simulink model "IEEE123bus_v2019b_Discrete"  (R2019b)
settings: Solver=ode4  StartTime=0.0  StopTime=5  FixedStep=Ts  MaxStep=1e-4  RelTol=1e-3
InitFcn:
  | a=1; % Loading Factor
  | Ts=50e-6;
  | % phase to sequence conversion of RXB matrices
  | c=1*exp(sqrt(-1)*(120*pi/180));
  | T=[1 1 1;1 c*c c;1 c c*c];
  | Tinv=1/3*[1 1 1;1 c c*c;1 c*c c];
  | 
  | % Simulation data for the IEEE 123 Node Test Feeder model
  | mi2km = 1.60934;%  miles to km conversion
  | ft2km = 0.0003048; % feet to km conversion
  | ms2F = 1*1e-6/(2*pi*60);% microsiemens to Farads conversion
  | 
  | %% Configuration 1
  | % Series Resitance and Reactance - ohm/mile
  | R_1 = [0.4576 0.1560 0.1535;0.1560 0.4666 0.1580;0.1535 0.1580 0.4615];
  | X_1 = [1.0780 0.5017 0.3849;0.5017 1.0482 0.4236;0.3849 0.4236 1.0651];
  | % charging susceptance - microsiemens/mile
  | B_1 = [5.6765 -1.8319 -0.6982;-1.8319 5.9809 -1.1645;-0.6982 -1.1645 5.3971];
  | 
  | R_1 = R_1/mi2km;
  | Rseq=Tinv*R_1*T;
  | R1_1=Rseq(2,2);R0_1=Rseq(1,1);
  | 
  | L_1 = (X_1/(2*pi*60))/mi2km;
  | Lseq=Tinv*L_1*T;
  | L1_1=Lseq(2,2);L0_1=Lseq(1,1);
  | 
  | C_1 =(B_1*ms2F)/mi2km;
  | Cseq=Tinv*C_1*T;
  | C1_1=Cseq(2,2);C0_1=Cseq(1,1);
  | %% Configuration 2 - series reactance - ohm/mile
  | R_2 = [0.4666 0.1580 0.1560;0.1580 0.4615 0.1535;0.1560 0.1535 0.4576];
  | X_2 = [1.0482 0.4236 0.5017;0.4236 1.0651 0.3849;0.5017 0.3849 1.0780];
  | % charging susceptance - microsiemens/mile
  | B_2 = [5.9809 -1.1645 -1.8319;-1.1645 5.3971 -0.6982;-1.8319 -0.6982 5.6765];
  | 
  | R_2 = R_2/mi2km;
  | Rseq=Tinv*R_2*T;
  | R1_2=Rseq(2,2);R0_2=Rseq(1,1);
  | 
  | L_2 = (X_2/(2*pi*60))/mi2km;
  | Lseq=Tinv*L_2*T;
  | L1_2=Lseq(2,2);L0_2=Lseq(1,1);
  | 
  | C_2 =(B_2*ms2F)/mi2km;
  | Cseq=Tinv*C_2*T;
  | C1_2=Cseq(2,2);C0_2=Cseq(1,1);
  | %% Configuration 3 - series reactance - ohm/mile
  | R_3 = [0.4615 0.1535 0.1580;0.1535 0.4576 0.1560;0.1580 0.1560 0.4666];
  | X_3 = [1.0651 0.3849 0.4236;0.3849 1.0780 0.5017;0.4236 0.5017 1.0482];
  | % charging susceptance - microsiemens/mile
  | B_3 = [5.3971 -0.6982 -1.1645;-0.6982 5.6765 -1.8319; -1.1645 -1.8319 5.9809];
  | 
  | R_3 = R_3/mi2km;
  | Rseq=Tinv*R_3*T;
  | R1_3=Rseq(2,2);R0_3=Rseq(1,1);
  | 
  | L_3 = (X_3/(2*pi*60))/mi2km;
  | Lseq=Tinv*L_3*T;
  | L1_3=Lseq(2,2);L0_3=Lseq(1,1);
  | 
  | C_3 =(B_3*ms2F)/mi2km;
  | Cseq=Tinv*C_3*T;
  | C1_3=Cseq(2,2);C0_3=Cseq(1,1);
  | %% Configuration 4 - series reactance - ohm/mile
  | R_4 = [0.4615 0.1580 0.1535;0.1580 0.4666 0.1560;0.1535 0.1560 0.4576];
  | X_4 = [1.0651 0.4236 0.3849;0.4236 1.0482 0.5017;0.3849 0.5017 1.0780];
  | % charging susceptance - microsiemens/mile
  | B_4 = [5.3971 -1.1645 -0.6982;-1.1645 5.9809 -1.8319;-0.6982 -1.8319 5.6765];
  | 
  | R_4 = R_4/mi2km;
  | Rseq=Tinv*R_4*T;
  | R1_4=Rseq(2,2);R0_4=Rseq(1,1);
  | 
  | L_4 = (X_4/(2*pi*60))/mi2km;
  | Lseq=Tinv*L_4*T;
  | L1_4=Lseq(2,2);L0_4=Lseq(1,1);
  | 
  | C_4 =(B_4*ms2F)/mi2km;
  | Cseq=Tinv*C_4*T;
  | C1_4=Cseq(2,2);C0_4=Cseq(1,1);
  | %% Configuration 5 - series reactance - ohm/mile
  | R_5 = [0.4666 0.1560 0.1580;0.1560 0.4576 0.1535;0.1580 0.1535 0.4615];
  | X_5 = [1.0482 0.5017 0.4236;0.5017 1.0780 0.3849;0.4236 0.3849 1.0651];
  | % charging susceptance - microsiemens/mile
  | B_5 = [5.9809 -1.8319 -1.1645;-1.8319 5.6765 -0.6982;-1.1645 -0.6982 5.3971];
  | 
  | R_5 = R_5/mi2km;
  | Rseq=Tinv*R_5*T;
  | R1_5=Rseq(2,2);R0_5=Rseq(1,1);
  | 
  | L_5 = (X_5/(2*pi*60))/mi2km;
  | Lseq=Tinv*L_5*T;
  | L1_5=Lseq(2,2);L0_5=Lseq(1,1);
  | 
  | C_5 =(B_5*ms2F)/mi2km;
  | Cseq=Tinv*C_5*T;
  | C1_5=Cseq(2,2);C0_5=Cseq(1,1);
  | %% Configuration 6 - series reactance - ohm/mile
  | R_6 = [0.4576 0.1535 0.1560;0.1535 0.4615 0.1580;0.1560 0.1580 0.4666];
  | X_6 = [1.0780 0.3849 0.5017;0.3849 1.0651 0.4236;0.5017 0.4236 1.0482];
  | % charging susceptance - microsiemens/mile
  | B_6 = [5.6765 -0.6982 -1.8319;-0.6982 5.3971 -1.1645;-1.8319 -1.1645 5.9809];
  | 
  | R_6 = R_6/mi2km;
  | Rseq=Tinv*R_6*T;
  | R1_6=Rseq(2,2);R0_6=Rseq(1,1);
  | 
  | L_6 = (X_6/(2*pi*60))/mi2km;
  | Lseq=Tinv*L_6*T;
  | L1_6=Lseq(2,2);L0_6=Lseq(1,1);
  | 
  | C_6 =(B_6*ms2F)/mi2km;
  | Cseq=Tinv*C_6*T;
  | C1_6=Cseq(2,2);C0_6=Cseq(1,1);
  | %% Configuration 7 - series reactance - ohm/mile
  | R_7 = [0.4576 0.0000 0.1535;0.0000 0.0000 0.0000;0.1535 0.0000 0.4615];
  | X_7 = [1.0780 0.0000 0.3849;0.0000 0.0000 0.0000;0.3849 0.0000 1.0651];
  | % charging susceptance - microsiemens/mile
  | B_7 = [5.1154 0.0000 -1.0549;0.0000 0.0000 0.0000;-1.0549 0.0000 5.1704];
  | 
  | R_7 = R_7/mi2km;
  | Rseq=Tinv*R_7*T;
  | R1_7=Rseq(2,2);R0_7=Rseq(1,1);
  | 
  | L_7 = (X_7/(2*pi*60))/mi2km;
  | Lseq=Tinv*L_7*T;
  | L1_7=Lseq(2,2);L0_7=Lseq(1,1);
  | 
  | C_7 =(B_7*ms2F)/mi2km;
  | Cseq=Tinv*C_7*T;
  | C1_7=Cseq(2,2);C0_7=Cseq(1,1);
  | %% Configuration 8 - series reactance - ohm/mile
  | R_8 = [0.4576 0.1535 0.0000;0.1535 0.4615 0.0000;0.0000 0.0000 0.0000];
  | X_8 = [1.0780 0.3849 0.0000;0.3849 1.0651 0.0000;0.0000 0.0000 0.0000];
  | % charging susceptance - microsiemens/mile
  | B_8 = [5.1154 -1.0549 0.0000;-1.0549 5.1704 0.0000;0.0000 0.0000 0.0000];
  | 
  | R_8 = R_8/mi2km;
  | Rseq=Tinv*R_8*T;
  | R1_8=Rseq(2,2);R0_8=Rseq(1,1);
  | 
  | L_8 = (X_8/(2*pi*60))/mi2km;
  | Lseq=Tinv*L_8*T;
  | L1_8=Lseq(2,2);L0_8=Lseq(1,1);
  | 
  | C_8 =(B_8*ms2F)/mi2km;
  | Cseq=Tinv*C_8*T;
  | C1_8=Cseq(2,2);C0_8=Cseq(1,1);
  | %% Configuration 9 - series reactance - ohm/mile
  | R_9 = [1.3292 0 0;0 0 0;0 0 0];
  | X_9 = [1.3475 0 0;0 0 0;0 0 0];
  | % charging susceptance - microsiemens/mile
  | B_9 = [4.5193 0 0;0 0 0;0 0 0];
  | 
  | R_9 = R_9/mi2km;
  | Rseq=Tinv*R_9*T;
  | R1_9=Rseq(2,2);R0_9=Rseq(1,1);
  | 
  | L_9 = (X_9/(2*pi*60))/mi2km;
  | Lseq=Tinv*L_9*T;
  | L1_9=Lseq(2,2);L0_9=Lseq(1,1);
  | 
  | C_9 =(B_9*ms2F)/mi2km;
  | Cseq=Tinv*C_9*T;
  | C1_9=Cseq(2,2);C0_9=Cseq(1,1);
  | %% Configuration 10- series reactance - ohm/mile
  | R_10 = [0 0 0;0 1.3292 0;0 0 0];
  | X_10 = [0 0 0;0 1.3475 0;0 0 0];
  | % charging susceptance - microsiemens/mile
  | B_10 = [0 0 0;0 4.5193 0;0 0 0];
  | 
  | R_10 = R_10/mi2km;
  | Rseq=Tinv*R_10*T;
  | R1_10=Rseq(2,2);R0_10=Rseq(1,1);
  | 
  | L_10 = (X_10/(2*pi*60))/mi2km;
  | Lseq=Tinv*L_10*T;
  | L1_10=Lseq(2,2);L0_10=Lseq(1,1);
  | 
  | C_10 =(B_10*ms2F)/mi2km;
  | Cseq=Tinv*C_10*T;
  | C1_10=Cseq(2,2);C0_10=Cseq(1,1);
  | %% Configuration 11 - series reactance - ohm/mile
  | R_11 = [0 0 0;0 0 0;0 0 1.3292];
  | X_11 = [0 0 0;0 0 0;0 0 1.3475];
  | % charging susceptance - microsiemens/mile
  | B_11 = [0 0 0;0 0 0;0 0 4.5193];
  | 
  | R_11 = R_11/mi2km;
  | Rseq=Tinv*R_11*T;
  | R1_11=Rseq(2,2);R0_11=Rseq(1,1);
  | 
  | L_11 = (X_11/(2*pi*60))/mi2km;
  | Lseq=Tinv*L_11*T;
  | L1_11=Lseq(2,2);L0_11=Lseq(1,1);
  | 
  | C_11 =(B_11*ms2F)/mi2km;
  | Cseq=Tinv*C_11*T;
  | C1_11=Cseq(2,2);C0_11=Cseq(1,1);
  | %% Configuration 12 - series reactance - ohm/mile
  | R_12 = [1.5209 0.5198 0.4924;0.5198 1.5329 0.5198;0.4924 0.5198 1.5209];
  | X_12 = [0.7521 0.2775 0.2157;0.2775 0.7162 0.2775;0.2157 0.2775 0.7521];
  | % charging susceptance - microsiemens/mile
  | B_12 = [67.2242 0.0000 0.0000;0.0000 67.2242 0.0000;0.0000 0.0000 67.2242];
  | 
  | R_12 = R_12/mi2km;
  | Rseq=Tinv*R_12*T;
  | R1_12=Rseq(2,2);R0_12=Rseq(1,1);
  | 
  | L_12 = (X_12/(2*pi*60))/mi2km;
  | Lseq=Tinv*L_12*T;
  | L1_12=Lseq(2,2);L0_12=Lseq(1,1);
  | 
  | C_12 =(B_12*ms2F)/mi2km;
  | Cseq=Tinv*C_12*T;
  | C1_12=Cseq(2,2);C0_12=Cseq(1,1);
undefined symbols (not defined in the file): D1, Delta, find_system
libraries: powerlib x768, powerlib_meascontrol x39
(part 1 of 6)
settings Model: ARTEMISmethode_block_infos=$$__separator__$$pi123variableloadwith3PV/ARTEMIS Guide$$__separator__$$  Creator=Arun  LastModifiedBy=USARSUR
settings DataIOCC: ReturnWorkspaceOutputs=off
settings DebuggingCC: UnconnectedInputMsg=none  UnconnectedOutputMsg=none  UnconnectedLineMsg=none  ArithmeticOperatorsInVariantConditions=warning
settings SFSimCC: SimUseLocalCustomCode=off  CustomCodeUndefinedFunction=UseInterfaceOnly
settings RTWCC: RTWUseLocalCustomCode=off
settings CodeAppCC: StateflowObjectComments=on
settings SimscapeCC: SimscapeNormalizeSystem=off

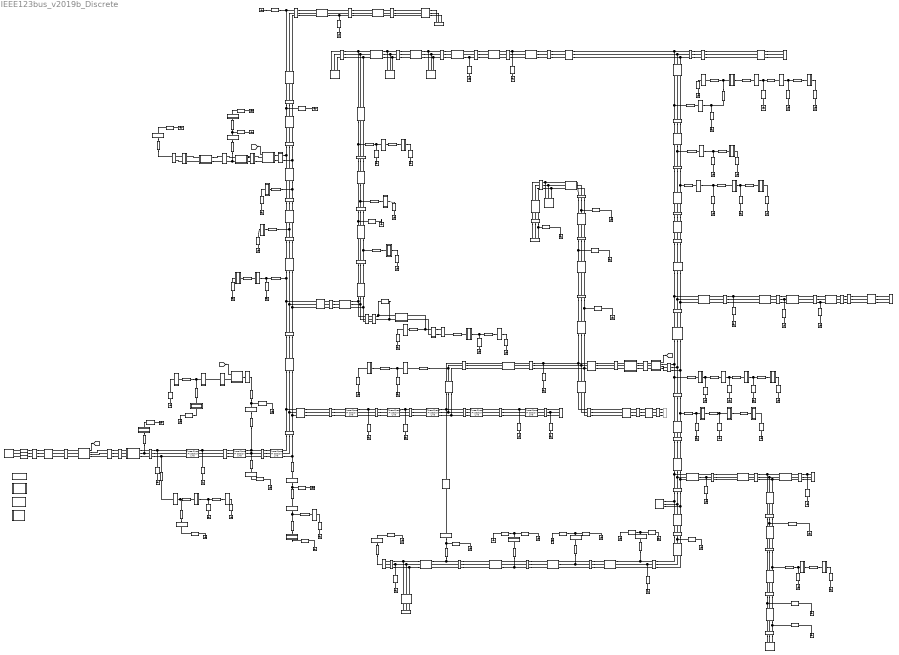
== system IEEE123bus_v2019b_Discrete ==
  note: Please consider citing following papers if the model was useful for your research
      |
      | A. Suresh, R. Bisht and S. Kamalasadan, "A Coordinated Control Architecture With Inverter-Based Resources and Legacy
      | Controllers of Power Distribution System for Voltage Profile Balance," in IEEE Transactions on Industry Applications, vol. 58,
      | no. 5, pp. 6701-6712, Sept.-Oct. 2022, doi: 10.1109/TIA.2022.3183030.
      |
      | A. Suresh, R. Bisht and S. Kamalasadan, "ADMM Based LQR for Voltage Regulation Using Distributed Energy Resources,"
      | 2020 IEEE International Conference on Power Electronics, Drives and Energy Systems (PEDES), 2020, pp. 1-6,
      | doi: 10.1109/PEDES49360.2020.9379625.
  note: Model Created by
      | Arun Suresh, Dr. Sukumar Kamalasadan,
      | University of North Carolina, Charlotte
  1 : powerlib/Measurements/Three-Phase V-I Measurement  VoltageMeasurement=phase-to-ground  SetLabelV=on  LabelV=V1  Vpu=off  VpuLL=off  CurrentMeasurement=no  SetLabelI=on  LabelI=I800  Ipu=off  Pbase=100e6  Vbase=24900  OutputType=Complex  PhasorSimulation=on  PSBequivalent=0
      settings: SourceProductName=Simscape Electrical
  1 Y PQ : powerlib/Elements/Series RLC Load  LConnTagsString=a  RConnTagsString=__new0  NominalVoltage=1.0*2401.78  NominalFrequency=60  ActivePower=40e3*a  InductivePower=20e3*a  CapacitivePower=0  Setx0=off  InitialVoltage=0  SetiL0=off  InitialCurrent=0  Measurements=None  LoadType=constant PQ
      settings: SourceProductName=Simscape Electrical
  1-2 10 : powerlib/Elements/Pi Section Line  LConnTagsString=__new0  RConnTagsString=__new0  Frequency=60  Resistance=R1_10  Inductance=L1_10  Capacitance=C1_10  Length=175*ft2km  PiSections=1  Measurements=None
      settings: AttributesFormatString=\n  SourceProductName=Simscape Electrical  SourceProductBaseCode=PS
  1-3 11 : powerlib/Elements/Pi Section Line  LConnTagsString=__new0  RConnTagsString=__new0  Frequency=60  Resistance=R1_11  Inductance=L1_11  Capacitance=C1_11  Length=250*ft2km  PiSections=1  Measurements=None
      settings: AttributesFormatString=\n  SourceProductName=Simscape Electrical  SourceProductBaseCode=PS
  1-7 1 : powerlib/Elements/Three-Phase PI Section Line  LConnTagsString=a|b|c  RConnTagsString=A|B|C  Frequency=60  Resistances=[R1_1 R0_1]  Inductances=[L1_1 L0_1]  Capacitances=[C1_1 C0_1]  Length=300*ft2km
      settings: SourceProductName=Simscape Electrical
  10 : Subsystem
  10 Y I : powerlib/Elements/Series RLC Load  LConnTagsString=a  RConnTagsString=__new0  NominalVoltage=1.0*2401.78  NominalFrequency=60  ActivePower=20e3*a  InductivePower=10e3*a  CapacitivePower=0  Setx0=off  InitialVoltage=0  SetiL0=off  InitialCurrent=0  Measurements=None  LoadType=constant I
      settings: SourceProductName=Simscape Electrical
  100 : powerlib/Measurements/Three-Phase V-I Measurement  VoltageMeasurement=phase-to-ground  SetLabelV=on  LabelV=V100  Vpu=off  VpuLL=off  CurrentMeasurement=no  SetLabelI=on  LabelI=I65  Ipu=off  Pbase=100e6  Vbase=24900  OutputType=Complex  PhasorSimulation=on  PSBequivalent=0
      settings: SourceProductName=Simscape Electrical
  100 Y Z : powerlib/Elements/Series RLC Load  LConnTagsString=a  RConnTagsString=__new0  NominalVoltage=1.0*2401.78  NominalFrequency=60  ActivePower=40e3*a  InductivePower=20e3*a  CapacitivePower=0  Setx0=off  InitialVoltage=0  SetiL0=off  InitialCurrent=0  Measurements=None  LoadType=constant Z
      settings: SourceProductName=Simscape Electrical
  100-450 3 : powerlib/Elements/Three-Phase PI Section Line  LConnTagsString=a|b|c  RConnTagsString=A|B|C  Frequency=60  Resistances=[R1_3 R0_3]  Inductances=[L1_3 L0_3]  Capacitances=[C1_3 C0_3]  Length=800*ft2km
      settings: SourceProductName=Simscape Electrical
  101 : powerlib/Measurements/Three-Phase V-I Measurement  VoltageMeasurement=phase-to-ground  SetLabelV=on  LabelV=V101  Vpu=off  VpuLL=off  CurrentMeasurement=no  SetLabelI=on  LabelI=I65  Ipu=off  Pbase=100e6  Vbase=24900  OutputType=Complex  PhasorSimulation=on  PSBequivalent=0
      settings: SourceProductName=Simscape Electrical
  101-102 11 : powerlib/Elements/Pi Section Line  LConnTagsString=__new0  RConnTagsString=__new0  Frequency=60  Resistance=R1_11  Inductance=L1_11  Capacitance=C1_11  Length=225*ft2km  PiSections=1  Measurements=None
      settings: AttributesFormatString=\n  SourceProductName=Simscape Electrical  SourceProductBaseCode=PS
  101-105 3 : powerlib/Elements/Three-Phase PI Section Line  LConnTagsString=a|b|c  RConnTagsString=A|B|C  Frequency=60  Resistances=[R1_3 R0_3]  Inductances=[L1_3 L0_3]  Capacitances=[C1_3 C0_3]  Length=275*ft2km
      settings: SourceProductName=Simscape Electrical
  102 : Subsystem
  102 Y Z : powerlib/Elements/Series RLC Load  LConnTagsString=a  RConnTagsString=__new0  NominalVoltage=1.0*2401.78  NominalFrequency=60  ActivePower=20e3*a  InductivePower=10e3*a  CapacitivePower=0  Setx0=off  InitialVoltage=0  SetiL0=off  InitialCurrent=0  Measurements=None  LoadType=constant Z
      settings: SourceProductName=Simscape Electrical
  102-103 11 : powerlib/Elements/Pi Section Line  LConnTagsString=__new0  RConnTagsString=__new0  Frequency=60  Resistance=R1_11  Inductance=L1_11  Capacitance=C1_11  Length=325*ft2km  PiSections=1  Measurements=None
      settings: AttributesFormatString=\n  SourceProductName=Simscape Electrical  SourceProductBaseCode=PS
  103 : Subsystem
  103 Y PQ : powerlib/Elements/Series RLC Load  LConnTagsString=a  RConnTagsString=__new0  NominalVoltage=1.0*2401.78  NominalFrequency=60  ActivePower=40e3*a  InductivePower=20e3*a  CapacitivePower=0  Setx0=off  InitialVoltage=0  SetiL0=off  InitialCurrent=0  Measurements=None  LoadType=constant PQ
      settings: SourceProductName=Simscape Electrical
  103-104 11 : powerlib/Elements/Pi Section Line  LConnTagsString=__new0  RConnTagsString=__new0  Frequency=60  Resistance=R1_11  Inductance=L1_11  Capacitance=C1_11  Length=700*ft2km  PiSections=1  Measurements=None
      settings: AttributesFormatString=\n  SourceProductName=Simscape Electrical  SourceProductBaseCode=PS
  104 : Subsystem
  104 Y PQ : powerlib/Elements/Series RLC Load  LConnTagsString=a  RConnTagsString=__new0  NominalVoltage=1.0*2401.78  NominalFrequency=60  ActivePower=40e3*a  InductivePower=20e3*a  CapacitivePower=0  Setx0=off  InitialVoltage=0  SetiL0=off  InitialCurrent=0  Measurements=None  LoadType=constant PQ
      settings: SourceProductName=Simscape Electrical
  105 : powerlib/Measurements/Three-Phase V-I Measurement  VoltageMeasurement=phase-to-ground  SetLabelV=on  LabelV=V105  Vpu=off  VpuLL=off  CurrentMeasurement=no  SetLabelI=on  LabelI=I65  Ipu=off  Pbase=100e6  Vbase=24900  OutputType=Complex  PhasorSimulation=on  PSBequivalent=0
      settings: SourceProductName=Simscape Electrical
  105-106 10 : powerlib/Elements/Pi Section Line  LConnTagsString=__new0  RConnTagsString=__new0  Frequency=60  Resistance=R1_10  Inductance=L1_10  Capacitance=C1_10  Length=225*ft2km  PiSections=1  Measurements=None
      settings: AttributesFormatString=\n  SourceProductName=Simscape Electrical  SourceProductBaseCode=PS
  105-108 3 : powerlib/Elements/Three-Phase PI Section Line  LConnTagsString=a|b|c  RConnTagsString=A|B|C  Frequency=60  Resistances=[R1_3 R0_3]  Inductances=[L1_3 L0_3]  Capacitances=[C1_3 C0_3]  Length=325*ft2km
      settings: SourceProductName=Simscape Electrical
  106 : Subsystem
  106 Y PQ : powerlib/Elements/Series RLC Load  LConnTagsString=a  RConnTagsString=__new0  NominalVoltage=1.0*2401.78  NominalFrequency=60  ActivePower=40e3*a  InductivePower=20e3*a  CapacitivePower=0  Setx0=off  InitialVoltage=0  SetiL0=off  InitialCurrent=0  Measurements=None  LoadType=constant PQ
      settings: SourceProductName=Simscape Electrical
  106-107 10 : powerlib/Elements/Pi Section Line  LConnTagsString=__new0  RConnTagsString=__new0  Frequency=60  Resistance=R1_10  Inductance=L1_10  Capacitance=C1_10  Length=575*ft2km  PiSections=1  Measurements=None
      settings: AttributesFormatString=\n  SourceProductName=Simscape Electrical  SourceProductBaseCode=PS
  107 : Subsystem
  107 Y PQ : powerlib/Elements/Series RLC Load  LConnTagsString=a  RConnTagsString=__new0  NominalVoltage=1.0*2401.78  NominalFrequency=60  ActivePower=40e3*a  InductivePower=20e3*a  CapacitivePower=0  Setx0=off  InitialVoltage=0  SetiL0=off  InitialCurrent=0  Measurements=None  LoadType=constant PQ
      settings: SourceProductName=Simscape Electrical
  108 : powerlib/Measurements/Three-Phase V-I Measurement  VoltageMeasurement=phase-to-ground  SetLabelV=on  LabelV=V108  Vpu=off  VpuLL=off  CurrentMeasurement=no  SetLabelI=on  LabelI=I65  Ipu=off  Pbase=100e6  Vbase=24900  OutputType=Complex  PhasorSimulation=on  PSBequivalent=0
      settings: SourceProductName=Simscape Electrical
  108-109 9 : powerlib/Elements/Pi Section Line  LConnTagsString=__new0  RConnTagsString=__new0  Frequency=60  Resistance=R1_9  Inductance=L1_9  Capacitance=C1_9  Length=450*ft2km  PiSections=1  Measurements=None
      settings: AttributesFormatString=\n  SourceProductName=Simscape Electrical  SourceProductBaseCode=PS
  108-300 3 : powerlib/Elements/Three-Phase PI Section Line  LConnTagsString=a|b|c  RConnTagsString=A|B|C  Frequency=60  Resistances=[R1_3 R0_3]  Inductances=[L1_3 L0_3]  Capacitances=[C1_3 C0_3]  Length=1000*ft2km
      settings: SourceProductName=Simscape Electrical
  109 : Subsystem
  109 Y PQ : powerlib/Elements/Series RLC Load  LConnTagsString=a  RConnTagsString=__new0  NominalVoltage=1.0*2401.78  NominalFrequency=60  ActivePower=40e3*a  InductivePower=20e3*a  CapacitivePower=0  Setx0=off  InitialVoltage=0  SetiL0=off  InitialCurrent=0  Measurements=None  LoadType=constant PQ
      settings: SourceProductName=Simscape Electrical
  109-110 9 : powerlib/Elements/Pi Section Line  LConnTagsString=__new0  RConnTagsString=__new0  Frequency=60  Resistance=R1_9  Inductance=L1_9  Capacitance=C1_9  Length=300*ft2km  PiSections=1  Measurements=None
      settings: AttributesFormatString=\n  SourceProductName=Simscape Electrical  SourceProductBaseCode=PS
  11 : Subsystem
  11 Y Z : powerlib/Elements/Series RLC Load  LConnTagsString=a  RConnTagsString=__new0  NominalVoltage=1.0*2401.78  NominalFrequency=60  ActivePower=40e3*a  InductivePower=20e3*a  CapacitivePower=0  Setx0=off  InitialVoltage=0  SetiL0=off  InitialCurrent=0  Measurements=None  LoadType=constant Z
      settings: SourceProductName=Simscape Electrical
  110 : Subsystem
  110-111 9 : powerlib/Elements/Pi Section Line  LConnTagsString=__new0  RConnTagsString=__new0  Frequency=60  Resistance=R1_9  Inductance=L1_9  Capacitance=C1_9  Length=575*ft2km  PiSections=1  Measurements=None
      settings: AttributesFormatString=\n  SourceProductName=Simscape Electrical  SourceProductBaseCode=PS
  110-112 9 : powerlib/Elements/Pi Section Line  LConnTagsString=__new0  RConnTagsString=__new0  Frequency=60  Resistance=R1_9  Inductance=L1_9  Capacitance=C1_9  Length=125*ft2km  PiSections=1  Measurements=None
      settings: AttributesFormatString=\n  SourceProductName=Simscape Electrical  SourceProductBaseCode=PS
  111 : Subsystem
  111 Y PQ : powerlib/Elements/Series RLC Load  LConnTagsString=a  RConnTagsString=__new0  NominalVoltage=1.0*2401.78  NominalFrequency=60  ActivePower=20e3*a  InductivePower=10e3*a  CapacitivePower=0  Setx0=off  InitialVoltage=0  SetiL0=off  InitialCurrent=0  Measurements=None  LoadType=constant PQ
      settings: SourceProductName=Simscape Electrical
  112 : Subsystem
  112 Y I : powerlib/Elements/Series RLC Load  LConnTagsString=a  RConnTagsString=__new0  NominalVoltage=1.0*2401.78  NominalFrequency=60  ActivePower=20e3*a  InductivePower=10e3*a  CapacitivePower=0  Setx0=off  InitialVoltage=0  SetiL0=off  InitialCurrent=0  Measurements=None  LoadType=constant I
      settings: SourceProductName=Simscape Electrical
  112-113 9 : powerlib/Elements/Pi Section Line  LConnTagsString=__new0  RConnTagsString=__new0  Frequency=60  Resistance=R1_9  Inductance=L1_9  Capacitance=C1_9  Length=525*ft2km  PiSections=1  Measurements=None
      settings: AttributesFormatString=\n  SourceProductName=Simscape Electrical  SourceProductBaseCode=PS
  113 : Subsystem
  113 Y Z : powerlib/Elements/Series RLC Load  LConnTagsString=a  RConnTagsString=__new0  NominalVoltage=1.0*2401.78  NominalFrequency=60  ActivePower=40e3*a  InductivePower=20e3*a  CapacitivePower=0  Setx0=off  InitialVoltage=0  SetiL0=off  InitialCurrent=0  Measurements=None  LoadType=constant PQ
      settings: SourceProductName=Simscape Electrical
  113-114 9 : powerlib/Elements/Pi Section Line  LConnTagsString=__new0  RConnTagsString=__new0  Frequency=60  Resistance=R1_9  Inductance=L1_9  Capacitance=C1_9  Length=325*ft2km  PiSections=1  Measurements=None
      settings: AttributesFormatString=\n  SourceProductName=Simscape Electrical  SourceProductBaseCode=PS
  114 : Subsystem
  114 Y PQ : powerlib/Elements/Series RLC Load  LConnTagsString=a  RConnTagsString=__new0  NominalVoltage=1.0*2401.78  NominalFrequency=60  ActivePower=20e3*a  InductivePower=10e3*a  CapacitivePower=0  Setx0=off  InitialVoltage=0  SetiL0=off  InitialCurrent=0  Measurements=None  LoadType=constant PQ
      settings: SourceProductName=Simscape Electrical
  12 : Subsystem
  12 Y PQ : powerlib/Elements/Series RLC Load  LConnTagsString=a  RConnTagsString=__new0  NominalVoltage=1.0*2401.78  NominalFrequency=60  ActivePower=20e3*a  InductivePower=10e3*a  CapacitivePower=0  Setx0=off  InitialVoltage=0  SetiL0=off  InitialCurrent=0  Measurements=None  LoadType=constant PQ
      settings: SourceProductName=Simscape Electrical
  13 : powerlib/Measurements/Three-Phase V-I Measurement  VoltageMeasurement=phase-to-ground  SetLabelV=on  LabelV=V13  Vpu=off  VpuLL=off  CurrentMeasurement=no  SetLabelI=on  LabelI=I800  Ipu=off  Pbase=100e6  Vbase=24900  OutputType=Complex  PhasorSimulation=on  PSBequivalent=0
      settings: SourceProductName=Simscape Electrical
  13-152 : powerlib/Elements/Three-Phase Breaker  InitialState=closed  SwitchA=off  SwitchB=off  SwitchC=off  SwitchTimes="[1/60  5/60]"  External=off  BreakerResistance=0.01  SnubberResistance=1e6  SnubberCapacitance=inf  Measurements=None
      settings: SourceProductName=Simscape Electrical
  13-18 2 : powerlib/Elements/Three-Phase PI Section Line  LConnTagsString=a|b|c  RConnTagsString=A|B|C  Frequency=60  Resistances=[R1_2 R0_2]  Inductances=[L1_2 L0_2]  Capacitances=[C1_2 C0_2]  Length=825*ft2km
      settings: SourceProductName=Simscape Electrical
  13-34 11 : powerlib/Elements/Pi Section Line  LConnTagsString=__new0  RConnTagsString=__new0  Frequency=60  Resistance=R1_11  Inductance=L1_11  Capacitance=C1_11  Length=150*ft2km  PiSections=1  Measurements=None
      settings: AttributesFormatString=\n  SourceProductName=Simscape Electrical  SourceProductBaseCode=PS
  135 : powerlib/Measurements/Three-Phase V-I Measurement  VoltageMeasurement=phase-to-ground  SetLabelV=on  LabelV=V135  Vpu=off  VpuLL=off  CurrentMeasurement=no  SetLabelI=on  LabelI=I800  Ipu=off  Pbase=100e6  Vbase=24900  OutputType=Complex  PhasorSimulation=on  PSBequivalent=0
      settings: SourceProductName=Simscape Electrical
  135-35 4 : powerlib/Elements/Three-Phase PI Section Line  LConnTagsString=a|b|c  RConnTagsString=A|B|C  Frequency=60  Resistances=[R1_4 R0_4]  Inductances=[L1_4 L0_4]  Capacitances=[C1_4 C0_4]  Length=375*ft2km
      settings: SourceProductName=Simscape Electrical
  14 : Subsystem
  14-10 9 : powerlib/Elements/Pi Section Line  LConnTagsString=__new0  RConnTagsString=__new0  Frequency=60  Resistance=R1_9  Inductance=L1_9  Capacitance=C1_9  Length=250*ft2km  PiSections=1  Measurements=None
      settings: AttributesFormatString=\n  SourceProductName=Simscape Electrical  SourceProductBaseCode=PS
  14-11 9 : powerlib/Elements/Pi Section Line  LConnTagsString=__new0  RConnTagsString=__new0  Frequency=60  Resistance=R1_9  Inductance=L1_9  Capacitance=C1_9  Length=250*ft2km  PiSections=1  Measurements=None
      settings: AttributesFormatString=\n  SourceProductName=Simscape Electrical  SourceProductBaseCode=PS
  149 : powerlib/Measurements/Three-Phase V-I Measurement  VoltageMeasurement=phase-to-ground  SetLabelV=on  LabelV=V149  Vpu=off  VpuLL=off  CurrentMeasurement=no  SetLabelI=on  LabelI=I800  Ipu=off  Pbase=100e6  Vbase=24900  OutputType=Complex  PhasorSimulation=on  PSBequivalent=0
      settings: SourceProductName=Simscape Electrical
  149-1 1 : Subsystem  mask(Three-Phase PI Section Block){Rl=R_1, Ll=L_1, Cl=C_1, L=400*ft2km}
      mask prompts: Rl "Resistance per unit Length(Ohm/Km)[3x3 matrix]"; Ll "Inductance per unit Length(H/Km)[3x3 matrix]"; Cl "Capacitance per unit Length(F/Km)[3x3 matrix]"; L "Length (Km)"
      mask help: This block models a three-phase transmission line with a single PI section.
  15 : Subsystem
  15-16 11 : powerlib/Elements/Pi Section Line  LConnTagsString=__new0  RConnTagsString=__new0  Frequency=60  Resistance=R1_11  Inductance=L1_11  Capacitance=C1_11  Length=375*ft2km  PiSections=1  Measurements=None
      settings: AttributesFormatString=\n  SourceProductName=Simscape Electrical  SourceProductBaseCode=PS
  15-17 11 : powerlib/Elements/Pi Section Line  LConnTagsString=__new0  RConnTagsString=__new0  Frequency=60  Resistance=R1_11  Inductance=L1_11  Capacitance=C1_11  Length=350*ft2km  PiSections=1  Measurements=None
      settings: AttributesFormatString=\n  SourceProductName=Simscape Electrical  SourceProductBaseCode=PS
  150 : powerlib/Measurements/Three-Phase V-I Measurement  VoltageMeasurement=phase-to-ground  SetLabelV=on  LabelV=V150  Vpu=off  VpuLL=off  CurrentMeasurement=yes  SetLabelI=on  LabelI=I150  Ipu=off  Pbase=100e6  Vbase=24900  OutputType=Complex  PhasorSimulation=on  PSBequivalent=0
      settings: SourceProductName=Simscape Electrical
  150-1 : powerlib/Elements/Three-Phase Breaker  InitialState=closed  SwitchA=off  SwitchB=off  SwitchC=off  SwitchTimes="[1/60  5/60]"  External=off  BreakerResistance=0.01  SnubberResistance=1e6  SnubberCapacitance=inf  Measurements=None
      settings: SourceProductName=Simscape Electrical
  151 : powerlib/Measurements/Three-Phase V-I Measurement  VoltageMeasurement=phase-to-ground  SetLabelV=on  LabelV=V151  Vpu=off  VpuLL=off  CurrentMeasurement=no  SetLabelI=on  LabelI=I65  Ipu=off  Pbase=100e6  Vbase=24900  OutputType=Complex  PhasorSimulation=on  PSBequivalent=0
      settings: SourceProductName=Simscape Electrical
  151-1 : powerlib/Elements/Three-Phase Breaker  InitialState=open  SwitchA=off  SwitchB=off  SwitchC=off  SwitchTimes="[1/60  5/60]"  External=off  BreakerResistance=0.01  SnubberResistance=1e6  SnubberCapacitance=inf  Measurements=None
      settings: SourceProductName=Simscape Electrical
  152 : powerlib/Measurements/Three-Phase V-I Measurement  VoltageMeasurement=phase-to-ground  SetLabelV=on  LabelV=V152  Vpu=off  VpuLL=off  CurrentMeasurement=no  SetLabelI=on  LabelI=I65  Ipu=off  Pbase=100e6  Vbase=24900  OutputType=Complex  PhasorSimulation=on  PSBequivalent=0
      settings: SourceProductName=Simscape Electrical
  152-52 1 : powerlib/Elements/Three-Phase PI Section Line  LConnTagsString=a|b|c  RConnTagsString=A|B|C  Frequency=60  Resistances=[R1_1 R0_1]  Inductances=[L1_1 L0_1]  Capacitances=[C1_1 C0_1]  Length=400*ft2km
      settings: SourceProductName=Simscape Electrical
  16 : Subsystem
  16 Y PQ : powerlib/Elements/Series RLC Load  LConnTagsString=a  RConnTagsString=__new0  NominalVoltage=1.0*2401.78  NominalFrequency=60  ActivePower=40e3*a  InductivePower=20e3*a  CapacitivePower=0  Setx0=off  InitialVoltage=0  SetiL0=off  InitialCurrent=0  Measurements=None  LoadType=constant PQ
      settings: SourceProductName=Simscape Electrical
  160 : powerlib/Measurements/Three-Phase V-I Measurement  VoltageMeasurement=phase-to-ground  SetLabelV=on  LabelV=V160  Vpu=off  VpuLL=off  CurrentMeasurement=no  SetLabelI=on  LabelI=I65  Ipu=off  Pbase=100e6  Vbase=24900  OutputType=Complex  PhasorSimulation=on  PSBequivalent=0
      settings: SourceProductName=Simscape Electrical
  160-67 6 : Subsystem  mask(Three-Phase PI Section Block){Rl=R_6, Ll=L_6, Cl=C_6, L=350*ft2km}
      mask prompts: Rl "Resistance per unit Length(Ohm/Km)[3x3 matrix]"; Ll "Inductance per unit Length(H/Km)[3x3 matrix]"; Cl "Capacitance per unit Length(F/Km)[3x3 matrix]"; L "Length (Km)"
      mask help: This block models a three-phase transmission line with a single PI section.
  17 : Subsystem
  17 Y PQ : powerlib/Elements/Series RLC Load  LConnTagsString=a  RConnTagsString=__new0  NominalVoltage=1.0*2401.78  NominalFrequency=60  ActivePower=20e3*a  InductivePower=10e3*a  CapacitivePower=0  Setx0=off  InitialVoltage=0  SetiL0=off  InitialCurrent=0  Measurements=None  LoadType=constant PQ
      settings: SourceProductName=Simscape Electrical
  18 : powerlib/Measurements/Three-Phase V-I Measurement  VoltageMeasurement=phase-to-ground  SetLabelV=on  LabelV=V18  Vpu=off  VpuLL=off  CurrentMeasurement=no  SetLabelI=on  LabelI=I800  Ipu=off  Pbase=100e6  Vbase=24900  OutputType=Complex  PhasorSimulation=on  PSBequivalent=0
      settings: SourceProductName=Simscape Electrical
  18-135 : powerlib/Elements/Three-Phase Breaker  InitialState=closed  SwitchA=off  SwitchB=off  SwitchC=off  SwitchTimes="[1/60  5/60]"  External=off  BreakerResistance=0.01  SnubberResistance=1e6  SnubberCapacitance=inf  Measurements=None
      settings: SourceProductName=Simscape Electrical
  18-19 9 : powerlib/Elements/Pi Section Line  LConnTagsString=__new0  RConnTagsString=__new0  Frequency=60  Resistance=R1_9  Inductance=L1_9  Capacitance=C1_9  Length=250*ft2km  PiSections=1  Measurements=None
      settings: AttributesFormatString=\n  SourceProductName=Simscape Electrical  SourceProductBaseCode=PS
  18-21 2 : powerlib/Elements/Three-Phase PI Section Line  LConnTagsString=a|b|c  RConnTagsString=A|B|C  Frequency=60  Resistances=[R1_2 R0_2]  Inductances=[L1_2 L0_2]  Capacitances=[C1_2 C0_2]  Length=300*ft2km
      settings: SourceProductName=Simscape Electrical
  19 : Subsystem
  19 Y PQ : powerlib/Elements/Series RLC Load  LConnTagsString=a  RConnTagsString=__new0  NominalVoltage=1.0*2401.78  NominalFrequency=60  ActivePower=40e3*a  InductivePower=20e3*a  CapacitivePower=0  Setx0=off  InitialVoltage=0  SetiL0=off  InitialCurrent=0  Measurements=None  LoadType=constant PQ
      settings: SourceProductName=Simscape Electrical
  19-20 9 : powerlib/Elements/Pi Section Line  LConnTagsString=__new0  RConnTagsString=__new0  Frequency=60  Resistance=R1_9  Inductance=L1_9  Capacitance=C1_9  Length=325*ft2km  PiSections=1  Measurements=None
      settings: AttributesFormatString=\n  SourceProductName=Simscape Electrical  SourceProductBaseCode=PS
  197 : powerlib/Measurements/Three-Phase V-I Measurement  VoltageMeasurement=phase-to-ground  SetLabelV=on  LabelV=V197  Vpu=off  VpuLL=off  CurrentMeasurement=no  SetLabelI=on  LabelI=I65  Ipu=off  Pbase=100e6  Vbase=24900  OutputType=Complex  PhasorSimulation=on  PSBequivalent=0
      settings: SourceProductName=Simscape Electrical
  197-101 3 : powerlib/Elements/Three-Phase PI Section Line  LConnTagsString=a|b|c  RConnTagsString=A|B|C  Frequency=60  Resistances=[R1_3 R0_3]  Inductances=[L1_3 L0_3]  Capacitances=[C1_3 C0_3]  Length=250*ft2km
      settings: SourceProductName=Simscape Electrical
  2 : Subsystem
  2 Y PQ : powerlib/Elements/Series RLC Load  LConnTagsString=a  RConnTagsString=__new0  NominalVoltage=1.0*2401.78  NominalFrequency=60  ActivePower=20e3*a  InductivePower=10e3*a  CapacitivePower=0  Setx0=off  InitialVoltage=0  SetiL0=off  InitialCurrent=0  Measurements=None  LoadType=constant PQ
      settings: SourceProductName=Simscape Electrical
  20 : Subsystem
  20 Y I : powerlib/Elements/Series RLC Load  LConnTagsString=a  RConnTagsString=__new0  NominalVoltage=1.0*2401.78  NominalFrequency=60  ActivePower=40e3*a  InductivePower=20e3*a  CapacitivePower=0  Setx0=off  InitialVoltage=0  SetiL0=off  InitialCurrent=0  Measurements=None  LoadType=constant I
      settings: SourceProductName=Simscape Electrical
  21 : powerlib/Measurements/Three-Phase V-I Measurement  VoltageMeasurement=phase-to-ground  SetLabelV=on  LabelV=V21  Vpu=off  VpuLL=off  CurrentMeasurement=no  SetLabelI=on  LabelI=I800  Ipu=off  Pbase=100e6  Vbase=24900  OutputType=Complex  PhasorSimulation=on  PSBequivalent=0
      settings: SourceProductName=Simscape Electrical
  21-22 10 : powerlib/Elements/Pi Section Line  LConnTagsString=__new0  RConnTagsString=__new0  Frequency=60  Resistance=R1_10  Inductance=L1_10  Capacitance=C1_10  Length=525*ft2km  PiSections=1  Measurements=None
      settings: AttributesFormatString=\n  SourceProductName=Simscape Electrical  SourceProductBaseCode=PS
  21-23 2 : powerlib/Elements/Three-Phase PI Section Line  LConnTagsString=a|b|c  RConnTagsString=A|B|C  Frequency=60  Resistances=[R1_2 R0_2]  Inductances=[L1_2 L0_2]  Capacitances=[C1_2 C0_2]  Length=250*ft2km
      settings: SourceProductName=Simscape Electrical
  22 : Subsystem
  22 Y Z : powerlib/Elements/Series RLC Load  LConnTagsString=a  RConnTagsString=__new0  NominalVoltage=1.0*2401.78  NominalFrequency=60  ActivePower=40e3*a  InductivePower=20e3*a  CapacitivePower=0  Setx0=off  InitialVoltage=0  SetiL0=off  InitialCurrent=0  Measurements=None  LoadType=constant Z
      settings: SourceProductName=Simscape Electrical
  23 : powerlib/Measurements/Three-Phase V-I Measurement  VoltageMeasurement=phase-to-ground  SetLabelV=on  LabelV=V23  Vpu=off  VpuLL=off  CurrentMeasurement=no  SetLabelI=on  LabelI=I800  Ipu=off  Pbase=100e6  Vbase=24900  OutputType=Complex  PhasorSimulation=on  PSBequivalent=0
      settings: SourceProductName=Simscape Electrical
  23-24 11 : powerlib/Elements/Pi Section Line  LConnTagsString=__new0  RConnTagsString=__new0  Frequency=60  Resistance=R1_11  Inductance=L1_11  Capacitance=C1_11  Length=550*ft2km  PiSections=1  Measurements=None
      settings: AttributesFormatString=\n  SourceProductName=Simscape Electrical  SourceProductBaseCode=PS
  23-25 2 : powerlib/Elements/Three-Phase PI Section Line  LConnTagsString=a|b|c  RConnTagsString=A|B|C  Frequency=60  Resistances=[R1_2 R0_2]  Inductances=[L1_2 L0_2]  Capacitances=[C1_2 C0_2]  Length=275*ft2km
      settings: SourceProductName=Simscape Electrical
  24 : Subsystem
  24 Y PQ : powerlib/Elements/Series RLC Load  LConnTagsString=a  RConnTagsString=__new0  NominalVoltage=1.0*2401.78  NominalFrequency=60  ActivePower=40e3*a  InductivePower=20e3*a  CapacitivePower=0  Setx0=off  InitialVoltage=0  SetiL0=off  InitialCurrent=0  Measurements=None  LoadType=constant PQ
      settings: SourceProductName=Simscape Electrical
  25 : powerlib/Measurements/Three-Phase V-I Measurement  VoltageMeasurement=phase-to-ground  SetLabelV=on  LabelV=V25  Vpu=off  VpuLL=off  CurrentMeasurement=no  SetLabelI=on  LabelI=I800  Ipu=off  Pbase=100e6  Vbase=24900  OutputType=Complex  PhasorSimulation=on  PSBequivalent=0
      settings: SourceProductName=Simscape Electrical
  25-26 7 : Subsystem  mask{Rl=R_7, Ll=L_7, Cl=C_7, L=350*ft2km}
      mask prompts: Rl "Resistance per unit Length(Ohm/Km)[3x3 matrix]"; Ll "Inductance per unit Length(H/Km)[3x3 matrix]"; Cl "Capacitance per unit Length(F/Km)[3x3 matrix"; L "Length (Km)"
      mask init:
      | W = sign(sum(abs(Rl)));
      | s = find(W==1);%Identify non zero rows and columns
      | 
      | Rt =Rl(s,s);
      | Rl= Rt;
      | Lt =Ll(s,s);
      | Ll= Lt;
      | Ct =Cl(s,s);
      | Cl= Ct;
  25-28 2 : powerlib/Elements/Three-Phase PI Section Line  LConnTagsString=a|b|c  RConnTagsString=A|B|C  Frequency=60  Resistances=[R1_2 R0_2]  Inductances=[L1_2 L0_2]  Capacitances=[C1_2 C0_2]  Length=200*ft2km
      settings: SourceProductName=Simscape Electrical
  250 : powerlib/Measurements/Three-Phase V-I Measurement  VoltageMeasurement=phase-to-ground  SetLabelV=on  LabelV=V250  Vpu=off  VpuLL=off  CurrentMeasurement=no  SetLabelI=on  LabelI=I800  Ipu=off  Pbase=100e6  Vbase=24900  OutputType=Complex  PhasorSimulation=on  PSBequivalent=0
      settings: SourceProductName=Simscape Electrical
  250-251 : powerlib/Elements/Three-Phase Breaker  InitialState=open  SwitchA=on  SwitchB=on  SwitchC=on  SwitchTimes="[1/60  5/60]"  External=off  BreakerResistance=0.01  SnubberResistance=1e6  SnubberCapacitance=inf  Measurements=None
      settings: SourceProductName=Simscape Electrical
  26 : Subsystem
  26-31 11 : powerlib/Elements/Pi Section Line  LConnTagsString=__new0  RConnTagsString=__new0  Frequency=60  Resistance=R1_11  Inductance=L1_11  Capacitance=C1_11  Length=225*ft2km  PiSections=1  Measurements=None
      settings: AttributesFormatString=\n  SourceProductName=Simscape Electrical  SourceProductBaseCode=PS
  26-7 7 : Subsystem  mask{Rl=R_7, Ll=L_7, Cl=C_7, L=275*ft2km}
      mask prompts: Rl "Resistance per unit Length(Ohm/Km)[3x3 matrix]"; Ll "Inductance per unit Length(H/Km)[3x3 matrix]"; Cl "Capacitance per unit Length(F/Km)[3x3 matrix"; L "Length (Km)"
      mask init:
      | W = sign(sum(abs(Rl)));
      | s = find(W==1);%Identify non zero rows and columns
      | 
      | Rt =Rl(s,s);
      | Rl= Rt;
      | Lt =Ll(s,s);
      | Ll= Lt;
      | Ct =Cl(s,s);
      | Cl= Ct;
  27 : Subsystem
  27-33 9 : powerlib/Elements/Pi Section Line  LConnTagsString=__new0  RConnTagsString=__new0  Frequency=60  Resistance=R1_9  Inductance=L1_9  Capacitance=C1_9  Length=500*ft2km  PiSections=1  Measurements=None
      settings: AttributesFormatString=\n  SourceProductName=Simscape Electrical  SourceProductBaseCode=PS
  28 : powerlib/Measurements/Three-Phase V-I Measurement  VoltageMeasurement=phase-to-ground  SetLabelV=on  LabelV=V28  Vpu=off  VpuLL=off  CurrentMeasurement=no  SetLabelI=on  LabelI=I800  Ipu=off  Pbase=100e6  Vbase=24900  OutputType=Complex  PhasorSimulation=on  PSBequivalent=0
      settings: SourceProductName=Simscape Electrical
  28 Y I : powerlib/Elements/Series RLC Load  LConnTagsString=a  RConnTagsString=__new0  NominalVoltage=1.0*2401.78  NominalFrequency=60  ActivePower=40e3*a  InductivePower=20e3*a  CapacitivePower=0  Setx0=off  InitialVoltage=0  SetiL0=off  InitialCurrent=0  Measurements=None  LoadType=constant I
      settings: SourceProductName=Simscape Electrical
  28-29 2 : powerlib/Elements/Three-Phase PI Section Line  LConnTagsString=a|b|c  RConnTagsString=A|B|C  Frequency=60  Resistances=[R1_2 R0_2]  Inductances=[L1_2 L0_2]  Capacitances=[C1_2 C0_2]  Length=300*ft2km
      settings: SourceProductName=Simscape Electrical
  29 : powerlib/Measurements/Three-Phase V-I Measurement  VoltageMeasurement=phase-to-ground  SetLabelV=on  LabelV=V29  Vpu=off  VpuLL=off  CurrentMeasurement=no  SetLabelI=on  LabelI=I800  Ipu=off  Pbase=100e6  Vbase=24900  OutputType=Complex  PhasorSimulation=on  PSBequivalent=0
      settings: SourceProductName=Simscape Electrical
  29 Y Z : powerlib/Elements/Series RLC Load  LConnTagsString=a  RConnTagsString=__new0  NominalVoltage=1.0*2401.78  NominalFrequency=60  ActivePower=40e3*a  InductivePower=20e3*a  CapacitivePower=0  Setx0=off  InitialVoltage=0  SetiL0=off  InitialCurrent=0  Measurements=None  LoadType=constant Z
      settings: SourceProductName=Simscape Electrical
  29-30 2 : powerlib/Elements/Three-Phase PI Section Line  LConnTagsString=a|b|c  RConnTagsString=A|B|C  Frequency=60  Resistances=[R1_2 R0_2]  Inductances=[L1_2 L0_2]  Capacitances=[C1_2 C0_2]  Length=350*ft2km
      settings: SourceProductName=Simscape Electrical
  3 : Subsystem
  3-4 11 : powerlib/Elements/Pi Section Line  LConnTagsString=__new0  RConnTagsString=__new0  Frequency=60  Resistance=R1_11  Inductance=L1_11  Capacitance=C1_11  Length=200*ft2km  PiSections=1  Measurements=None
      settings: AttributesFormatString=\n  SourceProductName=Simscape Electrical  SourceProductBaseCode=PS
  3-5 11 : powerlib/Elements/Pi Section Line  LConnTagsString=__new0  RConnTagsString=__new0  Frequency=60  Resistance=R1_11  Inductance=L1_11  Capacitance=C1_11  Length=325*ft2km  PiSections=1  Measurements=None
      settings: AttributesFormatString=\n  SourceProductName=Simscape Electrical  SourceProductBaseCode=PS
  "30 " : powerlib/Measurements/Three-Phase V-I Measurement  VoltageMeasurement=phase-to-ground  SetLabelV=on  LabelV=V30  Vpu=off  VpuLL=off  CurrentMeasurement=no  SetLabelI=on  LabelI=I800  Ipu=off  Pbase=100e6  Vbase=24900  OutputType=Complex  PhasorSimulation=on  PSBequivalent=0
      settings: SourceProductName=Simscape Electrical
  30 Y PQ : powerlib/Elements/Series RLC Load  LConnTagsString=a  RConnTagsString=__new0  NominalVoltage=1.0*2401.78  NominalFrequency=60  ActivePower=40e3*a  InductivePower=20e3*a  CapacitivePower=0  Setx0=off  InitialVoltage=0  SetiL0=off  InitialCurrent=0  Measurements=None  LoadType=constant PQ
      settings: SourceProductName=Simscape Electrical
  30-250 2 : powerlib/Elements/Three-Phase PI Section Line  LConnTagsString=a|b|c  RConnTagsString=A|B|C  Frequency=60  Resistances=[R1_2 R0_2]  Inductances=[L1_2 L0_2]  Capacitances=[C1_2 C0_2]  Length=200*ft2km
      settings: SourceProductName=Simscape Electrical
  300 : powerlib/Measurements/Three-Phase V-I Measurement  VoltageMeasurement=phase-to-ground  SetLabelV=on  LabelV=V300  Vpu=off  VpuLL=off  CurrentMeasurement=no  SetLabelI=on  LabelI=I65  Ipu=off  Pbase=100e6  Vbase=24900  OutputType=Complex  PhasorSimulation=on  PSBequivalent=0
      settings: SourceProductName=Simscape Electrical
  300-1 : powerlib/Elements/Three-Phase Breaker  InitialState=open  SwitchA=off  SwitchB=off  SwitchC=off  SwitchTimes="[1/60  5/60]"  External=off  BreakerResistance=0.01  SnubberResistance=1e6  SnubberCapacitance=inf  Measurements=None
      settings: SourceProductName=Simscape Electrical
  31 : Subsystem
  31 Y PQ : powerlib/Elements/Series RLC Load  LConnTagsString=a  RConnTagsString=__new0  NominalVoltage=1.0*2401.78  NominalFrequency=60  ActivePower=20e3*a  InductivePower=10e3*a  CapacitivePower=0  Setx0=off  InitialVoltage=0  SetiL0=off  InitialCurrent=0  Measurements=None  LoadType=constant PQ
      settings: SourceProductName=Simscape Electrical
  31-32 11 : powerlib/Elements/Pi Section Line  LConnTagsString=__new0  RConnTagsString=__new0  Frequency=60  Resistance=R1_11  Inductance=L1_11  Capacitance=C1_11  Length=300*ft2km  PiSections=1  Measurements=None
      settings: AttributesFormatString=\n  SourceProductName=Simscape Electrical  SourceProductBaseCode=PS
  32 : Subsystem
  32 Y PQ : powerlib/Elements/Series RLC Load  LConnTagsString=a  RConnTagsString=__new0  NominalVoltage=1.0*2401.78  NominalFrequency=60  ActivePower=20e3*a  InductivePower=10e3*a  CapacitivePower=0  Setx0=off  InitialVoltage=0  SetiL0=off  InitialCurrent=0  Measurements=None  LoadType=constant PQ
      settings: SourceProductName=Simscape Electrical
  33 : Subsystem
  33 Y I : powerlib/Elements/Series RLC Load  LConnTagsString=a  RConnTagsString=__new0  NominalVoltage=1.0*2401.78  NominalFrequency=60  ActivePower=40e3*a  InductivePower=20e3*a  CapacitivePower=0  Setx0=off  InitialVoltage=0  SetiL0=off  InitialCurrent=0  Measurements=None  LoadType=constant I
      settings: SourceProductName=Simscape Electrical
  34 : Subsystem
  34 Y Z : powerlib/Elements/Series RLC Load  LConnTagsString=a  RConnTagsString=__new0  NominalVoltage=1.0*2401.78  NominalFrequency=60  ActivePower=40e3*a  InductivePower=20e3*a  CapacitivePower=0  Setx0=off  InitialVoltage=0  SetiL0=off  InitialCurrent=0  Measurements=None  LoadType=constant Z
      settings: SourceProductName=Simscape Electrical
  34-15 11 : powerlib/Elements/Pi Section Line  LConnTagsString=__new0  RConnTagsString=__new0  Frequency=60  Resistance=R1_11  Inductance=L1_11  Capacitance=C1_11  Length=100*ft2km  PiSections=1  Measurements=None
      settings: AttributesFormatString=\n  SourceProductName=Simscape Electrical  SourceProductBaseCode=PS
  35 : powerlib/Measurements/Three-Phase V-I Measurement  VoltageMeasurement=phase-to-ground  SetLabelV=on  LabelV=V35  Vpu=off  VpuLL=off  CurrentMeasurement=no  SetLabelI=on  LabelI=I800  Ipu=off  Pbase=100e6  Vbase=24900  OutputType=Complex  PhasorSimulation=on  PSBequivalent=0
      settings: SourceProductName=Simscape Electrical
  35 D PQ : powerlib/Elements/Series RLC Load  LConnTagsString=a  RConnTagsString=__new0  NominalVoltage=1.0*4160  NominalFrequency=60  ActivePower=40e3*a  InductivePower=20e3*a  CapacitivePower=0  Setx0=off  InitialVoltage=0  SetiL0=off  InitialCurrent=0  Measurements=None  LoadType=constant I
      settings: SourceProductName=Simscape Electrical
  35-36 8 : Subsystem  mask(Three-Phase PI Section Block){Rl=R_8, Ll=L_8, Cl=C_8, L=650*ft2km}
      mask prompts: Rl "Resistance per unit Length(Ohm/Km)[3x3 matrix]"; Ll "Inductance per unit Length(H/Km)[3x3 matrix]"; Cl "Capacitance per unit Length(F/Km)[3x3 matrix"; L "Length (Km)"
      mask help: This block models a two-phase transmission line with a single PI section.
      mask init:
      | W = sign(sum(abs(Rl)));
      | s = find(W==1);%Identify non zero rows and columns
      | 
      | Rt =Rl(s,s);
      | Rl= Rt;
      | Lt =Ll(s,s);
      | Ll= Lt;
      | Ct =Cl(s,s);
      | Cl= Ct;
  35-40 1 : powerlib/Elements/Three-Phase PI Section Line  LConnTagsString=a|b|c  RConnTagsString=A|B|C  Frequency=60  Resistances=[R1_1 R0_1]  Inductances=[L1_1 L0_1]  Capacitances=[C1_1 C0_1]  Length=250*ft2km
      settings: SourceProductName=Simscape Electrical
  36 : Subsystem
  36-37 9 : powerlib/Elements/Pi Section Line  LConnTagsString=__new0  RConnTagsString=__new0  Frequency=60  Resistance=R1_9  Inductance=L1_9  Capacitance=C1_9  Length=300*ft2km  PiSections=1  Measurements=None
      settings: AttributesFormatString=\n  SourceProductName=Simscape Electrical  SourceProductBaseCode=PS
  36-38 10 : powerlib/Elements/Pi Section Line  LConnTagsString=__new0  RConnTagsString=__new0  Frequency=60  Resistance=R1_10  Inductance=L1_10  Capacitance=C1_10  Length=250*ft2km  PiSections=1  Measurements=None
      settings: AttributesFormatString=\n  SourceProductName=Simscape Electrical  SourceProductBaseCode=PS
  37 : Subsystem
  37 Y Z : powerlib/Elements/Series RLC Load  LConnTagsString=a  RConnTagsString=__new0  NominalVoltage=1.0*2401.78  NominalFrequency=60  ActivePower=40e3*a  InductivePower=20e3*a  CapacitivePower=0  Setx0=off  InitialVoltage=0  SetiL0=off  InitialCurrent=0  Measurements=None  LoadType=constant Z
      settings: SourceProductName=Simscape Electrical
  38 : Subsystem
  38 Y I : powerlib/Elements/Series RLC Load  LConnTagsString=a  RConnTagsString=__new0  NominalVoltage=1.0*2401.78  NominalFrequency=60  ActivePower=20e3*a  InductivePower=10e3*a  CapacitivePower=0  Setx0=off  InitialVoltage=0  SetiL0=off  InitialCurrent=0  Measurements=None  LoadType=constant I
      settings: SourceProductName=Simscape Electrical
  38-39 10 : powerlib/Elements/Pi Section Line  LConnTagsString=__new0  RConnTagsString=__new0  Frequency=60  Resistance=R1_10  Inductance=L1_10  Capacitance=C1_10  Length=325*ft2km  PiSections=1  Measurements=None
      settings: AttributesFormatString=\n  SourceProductName=Simscape Electrical  SourceProductBaseCode=PS
  39 : Subsystem
  39 Y PQ : powerlib/Elements/Series RLC Load  LConnTagsString=a  RConnTagsString=__new0  NominalVoltage=1.0*2401.78  NominalFrequency=60  ActivePower=20e3*a  InductivePower=10e3*a  CapacitivePower=0  Setx0=off  InitialVoltage=0  SetiL0=off  InitialCurrent=0  Measurements=None  LoadType=constant PQ
      settings: SourceProductName=Simscape Electrical
  4 : Subsystem
  40 : powerlib/Measurements/Three-Phase V-I Measurement  VoltageMeasurement=phase-to-ground  SetLabelV=on  LabelV=V40  Vpu=off  VpuLL=off  CurrentMeasurement=no  SetLabelI=on  LabelI=I800  Ipu=off  Pbase=100e6  Vbase=24900  OutputType=Complex  PhasorSimulation=on  PSBequivalent=0
      settings: SourceProductName=Simscape Electrical
  40-41 11 : powerlib/Elements/Pi Section Line  LConnTagsString=__new0  RConnTagsString=__new0  Frequency=60  Resistance=R1_11  Inductance=L1_11  Capacitance=C1_11  Length=325*ft2km  PiSections=1  Measurements=None
      settings: AttributesFormatString=\n  SourceProductName=Simscape Electrical  SourceProductBaseCode=PS
  40-42 1 : powerlib/Elements/Three-Phase PI Section Line  LConnTagsString=a|b|c  RConnTagsString=A|B|C  Frequency=60  Resistances=[R1_1 R0_1]  Inductances=[L1_1 L0_1]  Capacitances=[C1_1 C0_1]  Length=250*ft2km
      settings: SourceProductName=Simscape Electrical
  41 : Subsystem
  41 Y PQ : powerlib/Elements/Series RLC Load  LConnTagsString=a  RConnTagsString=__new0  NominalVoltage=1.0*2401.78  NominalFrequency=60  ActivePower=20e3*a  InductivePower=10e3*a  CapacitivePower=0  Setx0=off  InitialVoltage=0  SetiL0=off  InitialCurrent=0  Measurements=None  LoadType=constant PQ
      settings: SourceProductName=Simscape Electrical
  4160 V swing : powerlib/Electrical Sources/Three-Phase Source  InternalConnection=Yg  VoltagePhases=on  Voltage=120e3  PhaseAngle=0  Voltage_phases=[1.0 1.0 1.0]*4160/sqrt(3)  PhaseAngles_phases=[0 -120 120 ]  Frequency=60  NonIdealSource=off  SpecifyImpedance=on  Resistance=.0001  Inductance=16.58e-3  ShortCircuitLevel=10e6  BaseVoltage=4160  XRratio=4.67e4  BusType=swing  Pref=0  Qref=0  Prefabc=[4e6/3 4e6/3 4e6/3]  Qrefabc=[0 0 0]  Qmin="[-inf  -inf -inf]"  Qmax="[inf  inf inf]"
      settings: SourceProductName=Simscape Electrical
  42 : powerlib/Measurements/Three-Phase V-I Measurement  VoltageMeasurement=phase-to-ground  SetLabelV=on  LabelV=V42  Vpu=off  VpuLL=off  CurrentMeasurement=no  SetLabelI=on  LabelI=I800  Ipu=off  Pbase=100e6  Vbase=24900  OutputType=Complex  PhasorSimulation=on  PSBequivalent=0
      settings: SourceProductName=Simscape Electrical
  42 Y PQ : powerlib/Elements/Series RLC Load  LConnTagsString=a  RConnTagsString=__new0  NominalVoltage=1.0*2401.78  NominalFrequency=60  ActivePower=20e3*a  InductivePower=10e3*a  CapacitivePower=0  Setx0=off  InitialVoltage=0  SetiL0=off  InitialCurrent=0  Measurements=None  LoadType=constant PQ
      settings: SourceProductName=Simscape Electrical
  42-43 10 : powerlib/Elements/Pi Section Line  LConnTagsString=__new0  RConnTagsString=__new0  Frequency=60  Resistance=R1_10  Inductance=L1_10  Capacitance=C1_10  Length=500*ft2km  PiSections=1  Measurements=None
      settings: AttributesFormatString=\n  SourceProductName=Simscape Electrical  SourceProductBaseCode=PS
  42-44 1 : powerlib/Elements/Three-Phase PI Section Line  LConnTagsString=a|b|c  RConnTagsString=A|B|C  Frequency=60  Resistances=[R1_1 R0_1]  Inductances=[L1_1 L0_1]  Capacitances=[C1_1 C0_1]  Length=200*ft2km
      settings: SourceProductName=Simscape Electrical
  43 : Subsystem
  43 Y Z : powerlib/Elements/Series RLC Load  LConnTagsString=a  RConnTagsString=__new0  NominalVoltage=1.0*2401.78  NominalFrequency=60  ActivePower=40e3*a  InductivePower=20e3*a  CapacitivePower=0  Setx0=off  InitialVoltage=0  SetiL0=off  InitialCurrent=0  Measurements=None  LoadType=constant Z
      settings: SourceProductName=Simscape Electrical
  44 : powerlib/Measurements/Three-Phase V-I Measurement  VoltageMeasurement=phase-to-ground  SetLabelV=on  LabelV=V44  Vpu=off  VpuLL=off  CurrentMeasurement=no  SetLabelI=on  LabelI=I800  Ipu=off  Pbase=100e6  Vbase=24900  OutputType=Complex  PhasorSimulation=on  PSBequivalent=0
      settings: SourceProductName=Simscape Electrical
  44-45 9 : powerlib/Elements/Pi Section Line  LConnTagsString=__new0  RConnTagsString=__new0  Frequency=60  Resistance=R1_9  Inductance=L1_9  Capacitance=C1_9  Length=200*ft2km  PiSections=1  Measurements=None
      settings: AttributesFormatString=\n  SourceProductName=Simscape Electrical  SourceProductBaseCode=PS
  44-47 1 : powerlib/Elements/Three-Phase PI Section Line  LConnTagsString=a|b|c  RConnTagsString=A|B|C  Frequency=60  Resistances=[R1_1 R0_1]  Inductances=[L1_1 L0_1]  Capacitances=[C1_1 C0_1]  Length=250*ft2km
      settings: SourceProductName=Simscape Electrical
  45 : Subsystem
  45 Y I : powerlib/Elements/Series RLC Load  LConnTagsString=a  RConnTagsString=__new0  NominalVoltage=1.0*2401.78  NominalFrequency=60  ActivePower=20e3*a  InductivePower=10e3*a  CapacitivePower=0  Setx0=off  InitialVoltage=0  SetiL0=off  InitialCurrent=0  Measurements=None  LoadType=constant I
      settings: SourceProductName=Simscape Electrical
  45-46 9 : powerlib/Elements/Pi Section Line  LConnTagsString=__new0  RConnTagsString=__new0  Frequency=60  Resistance=R1_9  Inductance=L1_9  Capacitance=C1_9  Length=300*ft2km  PiSections=1  Measurements=None
      settings: AttributesFormatString=\n  SourceProductName=Simscape Electrical  SourceProductBaseCode=PS
  450 : powerlib/Measurements/Three-Phase V-I Measurement  VoltageMeasurement=phase-to-ground  SetLabelV=on  LabelV=V450  Vpu=off  VpuLL=off  CurrentMeasurement=no  SetLabelI=on  LabelI=I65  Ipu=off  Pbase=100e6  Vbase=24900  OutputType=Complex  PhasorSimulation=on  PSBequivalent=0
      settings: SourceProductName=Simscape Electrical
  450-451 : powerlib/Elements/Three-Phase Breaker  InitialState=open  SwitchA=off  SwitchB=off  SwitchC=off  SwitchTimes="[1/60  5/60]"  External=off  BreakerResistance=0.01  SnubberResistance=1e6  SnubberCapacitance=inf  Measurements=None
      settings: SourceProductName=Simscape Electrical
  46 : Subsystem
  46 Y PQ : powerlib/Elements/Series RLC Load  LConnTagsString=a  RConnTagsString=__new0  NominalVoltage=1.0*2401.78  NominalFrequency=60  ActivePower=20e3*a  InductivePower=10e3*a  CapacitivePower=0  Setx0=off  InitialVoltage=0  SetiL0=off  InitialCurrent=0  Measurements=None  LoadType=constant PQ
      settings: SourceProductName=Simscape Electrical
  47 : powerlib/Measurements/Three-Phase V-I Measurement  VoltageMeasurement=phase-to-ground  SetLabelV=on  LabelV=V47  Vpu=off  VpuLL=off  CurrentMeasurement=no  SetLabelI=on  LabelI=I800  Ipu=off  Pbase=100e6  Vbase=24900  OutputType=Complex  PhasorSimulation=on  PSBequivalent=0
      settings: SourceProductName=Simscape Electrical
  47 Y I : powerlib/Elements/Three-Phase Series RLC Load  LConnTagsString=A|B|C  Configuration=Y (grounded)  NominalVoltage=120e3  Vabc=[ 1.0 1.0 1.0]*2401.78  Vabcp=[1e3 1e3 1e3]  NominalFrequency=60  UnbalancedPower=on  ActivePower=1e+006  InductivePower=0  CapacitivePower=0  Pabc=[35 35 35 ]*1e3*a  QLabc=[25 25 25 ]*1e3*a  QCabc=[0 0 0]  Pabcp=[10e3 9e3 11e3]  QLabcp=[100 90 110]  QCabcp=[100 90 110]  Measurements=None  LoadType=constant I
      settings: SourceProductName=Simscape Electrical
  47-48 4 : powerlib/Elements/Three-Phase PI Section Line  LConnTagsString=a|b|c  RConnTagsString=A|B|C  Frequency=60  Resistances=[R1_4 R0_4]  Inductances=[L1_4 L0_4]  Capacitances=[C1_4 C0_4]  Length=150*ft2km
      settings: SourceProductName=Simscape Electrical
  47-49 4 : powerlib/Elements/Three-Phase PI Section Line  LConnTagsString=a|b|c  RConnTagsString=A|B|C  Frequency=60  Resistances=[R1_4 R0_4]  Inductances=[L1_4 L0_4]  Capacitances=[C1_4 C0_4]  Length=250*ft2km
      settings: SourceProductName=Simscape Electrical
  48 : powerlib/Measurements/Three-Phase V-I Measurement  VoltageMeasurement=phase-to-ground  SetLabelV=on  LabelV=V48  Vpu=off  VpuLL=off  CurrentMeasurement=no  SetLabelI=on  LabelI=I800  Ipu=off  Pbase=100e6  Vbase=24900  OutputType=Complex  PhasorSimulation=on  PSBequivalent=0
      settings: SourceProductName=Simscape Electrical
  48 Y Z : powerlib/Elements/Three-Phase Series RLC Load  LConnTagsString=A|B|C  Configuration=Y (grounded)  NominalVoltage=120e3  Vabc=[ 1.0 1.0 1.0]*2401.78  Vabcp=[1e3 1e3 1e3]  NominalFrequency=60  UnbalancedPower=on  ActivePower=1e+006  InductivePower=0  CapacitivePower=0  Pabc=[70 70 70]*1e3*a  QLabc=[50 50 50]*1e3*a  QCabc=[0 0 0]  Pabcp=[10e3 9e3 11e3]  QLabcp=[100 90 110]  QCabcp=[100 90 110]  Measurements=None  LoadType=constant Z
      settings: SourceProductName=Simscape Electrical
  49 : powerlib/Measurements/Three-Phase V-I Measurement  VoltageMeasurement=phase-to-ground  SetLabelV=on  LabelV=V49  Vpu=off  VpuLL=off  CurrentMeasurement=no  SetLabelI=on  LabelI=I800  Ipu=off  Pbase=100e6  Vbase=24900  OutputType=Complex  PhasorSimulation=on  PSBequivalent=0
      settings: SourceProductName=Simscape Electrical
  49 Y PQ : powerlib/Elements/Three-Phase Series RLC Load  LConnTagsString=A|B|C  Configuration=Y (grounded)  NominalVoltage=120e3  Vabc=[ 1.0 1.0 1.0]*2401.78  Vabcp=[1e3 1e3 1e3]  NominalFrequency=60  UnbalancedPower=on  ActivePower=1e+006  InductivePower=0  CapacitivePower=0  Pabc=[35 70 35]*1e3*a  QLabc=[25 50 20]*1e3*a  QCabc=[0 0 0]  Pabcp=[10e3 9e3 11e3]  QLabcp=[100 90 110]  QCabcp=[100 90 110]  Measurements=None  LoadType=constant PQ
      settings: SourceProductName=Simscape Electrical
  49-50 4 : powerlib/Elements/Three-Phase PI Section Line  LConnTagsString=a|b|c  RConnTagsString=A|B|C  Frequency=60  Resistances=[R1_4 R0_4]  Inductances=[L1_4 L0_4]  Capacitances=[C1_4 C0_4]  Length=250*ft2km
      settings: SourceProductName=Simscape Electrical
  4Y PQ : powerlib/Elements/Series RLC Load  LConnTagsString=a  RConnTagsString=__new0  NominalVoltage=1.0*2401.78  NominalFrequency=60  ActivePower=40e3*a  InductivePower=20e3*a  CapacitivePower=0  Setx0=off  InitialVoltage=0  SetiL0=off  InitialCurrent=0  Measurements=None  LoadType=constant PQ
      settings: SourceProductName=Simscape Electrical
  5 : Subsystem
  5 Y I : powerlib/Elements/Series RLC Load  LConnTagsString=a  RConnTagsString=__new0  NominalVoltage=1.0*2401.78  NominalFrequency=60  ActivePower=20e3*a  InductivePower=10e3*a  CapacitivePower=0  Setx0=off  InitialVoltage=0  SetiL0=off  InitialCurrent=0  Measurements=None  LoadType=constant I
      settings: SourceProductName=Simscape Electrical
  5-6 11 : powerlib/Elements/Pi Section Line  LConnTagsString=__new0  RConnTagsString=__new0  Frequency=60  Resistance=R1_11  Inductance=L1_11  Capacitance=C1_11  Length=250*ft2km  PiSections=1  Measurements=None
      settings: AttributesFormatString=\n  SourceProductName=Simscape Electrical  SourceProductBaseCode=PS
  50 : powerlib/Measurements/Three-Phase V-I Measurement  VoltageMeasurement=phase-to-ground  SetLabelV=on  LabelV=V50  Vpu=off  VpuLL=off  CurrentMeasurement=no  SetLabelI=on  LabelI=I800  Ipu=off  Pbase=100e6  Vbase=24900  OutputType=Complex  PhasorSimulation=on  PSBequivalent=0
      settings: SourceProductName=Simscape Electrical
  50 Y PQ : powerlib/Elements/Series RLC Load  LConnTagsString=a  RConnTagsString=__new0  NominalVoltage=1.0*2401.78  NominalFrequency=60  ActivePower=40e3*a  InductivePower=20e3*a  CapacitivePower=0  Setx0=off  InitialVoltage=0  SetiL0=off  InitialCurrent=0  Measurements=None  LoadType=constant PQ
      settings: SourceProductName=Simscape Electrical
  50-51 4 : powerlib/Elements/Three-Phase PI Section Line  LConnTagsString=a|b|c  RConnTagsString=A|B|C  Frequency=60  Resistances=[R1_4 R0_4]  Inductances=[L1_4 L0_4]  Capacitances=[C1_4 C0_4]  Length=250*ft2km
      settings: SourceProductName=Simscape Electrical
  51 : powerlib/Measurements/Three-Phase V-I Measurement  VoltageMeasurement=phase-to-ground  SetLabelV=on  LabelV=V51  Vpu=off  VpuLL=off  CurrentMeasurement=no  SetLabelI=on  LabelI=I800  Ipu=off  Pbase=100e6  Vbase=24900  OutputType=Complex  PhasorSimulation=on  PSBequivalent=0
      settings: SourceProductName=Simscape Electrical
  51 Y PQ : powerlib/Elements/Series RLC Load  LConnTagsString=a  RConnTagsString=__new0  NominalVoltage=1.0*2401.78  NominalFrequency=60  ActivePower=20e3*a  InductivePower=10e3*a  CapacitivePower=0  Setx0=off  InitialVoltage=0  SetiL0=off  InitialCurrent=0  Measurements=None  LoadType=constant PQ
      settings: SourceProductName=Simscape Electrical
  51-151 4 : powerlib/Elements/Three-Phase PI Section Line  LConnTagsString=a|b|c  RConnTagsString=A|B|C  Frequency=60  Resistances=[R1_4 R0_4]  Inductances=[L1_4 L0_4]  Capacitances=[C1_4 C0_4]  Length=500*ft2km
      settings: SourceProductName=Simscape Electrical
  52 : powerlib/Measurements/Three-Phase V-I Measurement  VoltageMeasurement=phase-to-ground  SetLabelV=on  LabelV=V52  Vpu=off  VpuLL=off  CurrentMeasurement=no  SetLabelI=on  LabelI=I65  Ipu=off  Pbase=100e6  Vbase=24900  OutputType=Complex  PhasorSimulation=on  PSBequivalent=0
      settings: SourceProductName=Simscape Electrical
  52 Y PQ : powerlib/Elements/Series RLC Load  LConnTagsString=a  RConnTagsString=__new0  NominalVoltage=1.0*2401.78  NominalFrequency=60  ActivePower=40e3*a  InductivePower=20e3*a  CapacitivePower=0  Setx0=off  InitialVoltage=0  SetiL0=off  InitialCurrent=0  Measurements=None  LoadType=constant PQ
      settings: SourceProductName=Simscape Electrical
  52-53 1 : powerlib/Elements/Three-Phase PI Section Line  LConnTagsString=a|b|c  RConnTagsString=A|B|C  Frequency=60  Resistances=[R1_1 R0_1]  Inductances=[L1_1 L0_1]  Capacitances=[C1_1 C0_1]  Length=200*ft2km
      settings: SourceProductName=Simscape Electrical
  53 : powerlib/Measurements/Three-Phase V-I Measurement  VoltageMeasurement=phase-to-ground  SetLabelV=on  LabelV=V53  Vpu=off  VpuLL=off  CurrentMeasurement=no  SetLabelI=on  LabelI=I65  Ipu=off  Pbase=100e6  Vbase=24900  OutputType=Complex  PhasorSimulation=on  PSBequivalent=0
      settings: SourceProductName=Simscape Electrical
  53 Y PQ : powerlib/Elements/Series RLC Load  LConnTagsString=a  RConnTagsString=__new0  NominalVoltage=1.0*2401.78  NominalFrequency=60  ActivePower=40e3*a  InductivePower=20e3*a  CapacitivePower=0  Setx0=off  InitialVoltage=0  SetiL0=off  InitialCurrent=0  Measurements=None  LoadType=constant PQ
      settings: SourceProductName=Simscape Electrical
  53-54 1 : powerlib/Elements/Three-Phase PI Section Line  LConnTagsString=a|b|c  RConnTagsString=A|B|C  Frequency=60  Resistances=[R1_1 R0_1]  Inductances=[L1_1 L0_1]  Capacitances=[C1_1 C0_1]  Length=125*ft2km
      settings: SourceProductName=Simscape Electrical
  54 : powerlib/Measurements/Three-Phase V-I Measurement  VoltageMeasurement=phase-to-ground  SetLabelV=on  LabelV=V54  Vpu=off  VpuLL=off  CurrentMeasurement=no  SetLabelI=on  LabelI=I65  Ipu=off  Pbase=100e6  Vbase=24900  OutputType=Complex  PhasorSimulation=on  PSBequivalent=0
      settings: SourceProductName=Simscape Electrical
  54-55 1 : powerlib/Elements/Three-Phase PI Section Line  LConnTagsString=a|b|c  RConnTagsString=A|B|C  Frequency=60  Resistances=[R1_1 R0_1]  Inductances=[L1_1 L0_1]  Capacitances=[C1_1 C0_1]  Length=275*ft2km
      settings: SourceProductName=Simscape Electrical
  54-57 3 : powerlib/Elements/Three-Phase PI Section Line  LConnTagsString=a|b|c  RConnTagsString=A|B|C  Frequency=60  Resistances=[R1_3 R0_3]  Inductances=[L1_3 L0_3]  Capacitances=[C1_3 C0_3]  Length=350*ft2km
      settings: SourceProductName=Simscape Electrical
  55 : powerlib/Measurements/Three-Phase V-I Measurement  VoltageMeasurement=phase-to-ground  SetLabelV=on  LabelV=V55  Vpu=off  VpuLL=off  CurrentMeasurement=no  SetLabelI=on  LabelI=I65  Ipu=off  Pbase=100e6  Vbase=24900  OutputType=Complex  PhasorSimulation=on  PSBequivalent=0
      settings: SourceProductName=Simscape Electrical
  55 Y Z : powerlib/Elements/Series RLC Load  LConnTagsString=a  RConnTagsString=__new0  NominalVoltage=1.0*2401.78  NominalFrequency=60  ActivePower=20e3*a  InductivePower=10e3*a  CapacitivePower=0  Setx0=off  InitialVoltage=0  SetiL0=off  InitialCurrent=0  Measurements=None  LoadType=constant Z
      settings: SourceProductName=Simscape Electrical
  55-56 1 : powerlib/Elements/Three-Phase PI Section Line  LConnTagsString=a|b|c  RConnTagsString=A|B|C  Frequency=60  Resistances=[R1_1 R0_1]  Inductances=[L1_1 L0_1]  Capacitances=[C1_1 C0_1]  Length=275*ft2km
      settings: SourceProductName=Simscape Electrical
  56 : powerlib/Measurements/Three-Phase V-I Measurement  VoltageMeasurement=phase-to-ground  SetLabelV=on  LabelV=V56  Vpu=off  VpuLL=off  CurrentMeasurement=no  SetLabelI=on  LabelI=I65  Ipu=off  Pbase=100e6  Vbase=24900  OutputType=Complex  PhasorSimulation=on  PSBequivalent=0
      settings: SourceProductName=Simscape Electrical
  56 Y PQ : powerlib/Elements/Series RLC Load  LConnTagsString=a  RConnTagsString=__new0  NominalVoltage=1.0*2401.78  NominalFrequency=60  ActivePower=20e3*a  InductivePower=10e3*a  CapacitivePower=0  Setx0=off  InitialVoltage=0  SetiL0=off  InitialCurrent=0  Measurements=None  LoadType=constant PQ
      settings: SourceProductName=Simscape Electrical
  57 : powerlib/Measurements/Three-Phase V-I Measurement  VoltageMeasurement=phase-to-ground  SetLabelV=on  LabelV=V57  Vpu=off  VpuLL=off  CurrentMeasurement=no  SetLabelI=on  LabelI=I65  Ipu=off  Pbase=100e6  Vbase=24900  OutputType=Complex  PhasorSimulation=on  PSBequivalent=0
      settings: SourceProductName=Simscape Electrical
  57-58 10 : powerlib/Elements/Pi Section Line  LConnTagsString=__new0  RConnTagsString=__new0  Frequency=60  Resistance=R1_10  Inductance=L1_10  Capacitance=C1_10  Length=250*ft2km  PiSections=1  Measurements=None
      settings: AttributesFormatString=\n  SourceProductName=Simscape Electrical  SourceProductBaseCode=PS
  57-60 3 : powerlib/Elements/Three-Phase PI Section Line  LConnTagsString=a|b|c  RConnTagsString=A|B|C  Frequency=60  Resistances=[R1_3 R0_3]  Inductances=[L1_3 L0_3]  Capacitances=[C1_3 C0_3]  Length=750*ft2km
      settings: SourceProductName=Simscape Electrical
  58 : Subsystem
  58 Y I : powerlib/Elements/Series RLC Load  LConnTagsString=a  RConnTagsString=__new0  NominalVoltage=1.0*2401.78  NominalFrequency=60  ActivePower=20e3*a  InductivePower=10e3*a  CapacitivePower=0  Setx0=off  InitialVoltage=0  SetiL0=off  InitialCurrent=0  Measurements=None  LoadType=constant I
      settings: SourceProductName=Simscape Electrical
  58-59 10 : powerlib/Elements/Pi Section Line  LConnTagsString=__new0  RConnTagsString=__new0  Frequency=60  Resistance=R1_10  Inductance=L1_10  Capacitance=C1_10  Length=10*ft2km  PiSections=1  Measurements=None
      settings: AttributesFormatString=\n  SourceProductName=Simscape Electrical  SourceProductBaseCode=PS
  59 : Subsystem
  59 Y PQ : powerlib/Elements/Series RLC Load  LConnTagsString=a  RConnTagsString=__new0  NominalVoltage=1.0*2401.78  NominalFrequency=60  ActivePower=20e3*a  InductivePower=10e3*a  CapacitivePower=0  Setx0=off  InitialVoltage=0  SetiL0=off  InitialCurrent=0  Measurements=None  LoadType=constant PQ
      settings: SourceProductName=Simscape Electrical
  59-94 : powerlib/Elements/Breaker  InitialState=0  SwitchingTimes="[1/60  5/60]"  External=off  BreakerResistance=0.01  SnubberResistance=1e6  SnubberCapacitance=inf  Measurements=None  MoreParameters=on  NoBreakLoop=off
      settings: SourceProductName=Simscape Electrical
  6 : Subsystem
  6 Y Z : powerlib/Elements/Series RLC Load  LConnTagsString=a  RConnTagsString=__new0  NominalVoltage=1.0*2401.78  NominalFrequency=60  ActivePower=40e3*a  InductivePower=20e3*a  CapacitivePower=0  Setx0=off  InitialVoltage=0  SetiL0=off  InitialCurrent=0  Measurements=None  LoadType=constant Z
      settings: SourceProductName=Simscape Electrical
  60 : powerlib/Measurements/Three-Phase V-I Measurement  VoltageMeasurement=phase-to-ground  SetLabelV=on  LabelV=V60  Vpu=off  VpuLL=off  CurrentMeasurement=no  SetLabelI=on  LabelI=I65  Ipu=off  Pbase=100e6  Vbase=24900  OutputType=Complex  PhasorSimulation=on  PSBequivalent=0
      settings: SourceProductName=Simscape Electrical
  60 Y PQ : powerlib/Elements/Series RLC Load  LConnTagsString=a  RConnTagsString=__new0  NominalVoltage=1.0*2401.78  NominalFrequency=60  ActivePower=20e3*a  InductivePower=10e3*a  CapacitivePower=0  Setx0=off  InitialVoltage=0  SetiL0=off  InitialCurrent=0  Measurements=None  LoadType=constant PQ
      settings: SourceProductName=Simscape Electrical
  60-1 : powerlib/Elements/Three-Phase Breaker  InitialState=closed  SwitchA=off  SwitchB=off  SwitchC=off  SwitchTimes="[1/60  5/60]"  External=off  BreakerResistance=0.01  SnubberResistance=1e6  SnubberCapacitance=inf  Measurements=None
      settings: SourceProductName=Simscape Electrical
  60-61 5 : powerlib/Elements/Three-Phase PI Section Line  LConnTagsString=a|b|c  RConnTagsString=A|B|C  Frequency=60  Resistances=[R1_5 R0_5]  Inductances=[L1_5 L0_5]  Capacitances=[C1_5 C0_5]  Length=550*ft2km
      settings: SourceProductName=Simscape Electrical
  60-62 12 : powerlib/Elements/Three-Phase PI Section Line  LConnTagsString=a|b|c  RConnTagsString=A|B|C  Frequency=60  Resistances=[R1_12 R0_12]  Inductances=[L1_12 L0_12]  Capacitances=[C1_12 C0_12]  Length=250*ft2km
      settings: SourceProductName=Simscape Electrical
  61 : powerlib/Measurements/Three-Phase V-I Measurement  VoltageMeasurement=phase-to-ground  SetLabelV=on  LabelV=V61  Vpu=off  VpuLL=off  CurrentMeasurement=no  SetLabelI=on  LabelI=I65  Ipu=off  Pbase=100e6  Vbase=24900  OutputType=Complex  PhasorSimulation=on  PSBequivalent=0
      settings: SourceProductName=Simscape Electrical
  61-610 : powerlib/Elements/Three-Phase Breaker  InitialState=closed  SwitchA=off  SwitchB=off  SwitchC=off  SwitchTimes="[1/60  5/60]"  External=off  BreakerResistance=0.01  SnubberResistance=1e6  SnubberCapacitance=inf  Measurements=None
      settings: SourceProductName=Simscape Electrical
  610 : powerlib/Measurements/Three-Phase V-I Measurement  VoltageMeasurement=phase-to-phase  SetLabelV=on  LabelV=V610  Vpu=off  VpuLL=off  CurrentMeasurement=no  SetLabelI=on  LabelI=I65  Ipu=off  Pbase=100e6  Vbase=24900  OutputType=Complex  PhasorSimulation=on  PSBequivalent=0
      settings: SourceProductName=Simscape Electrical
  62 : powerlib/Measurements/Three-Phase V-I Measurement  VoltageMeasurement=phase-to-ground  SetLabelV=on  LabelV=V62  Vpu=off  VpuLL=off  CurrentMeasurement=no  SetLabelI=on  LabelI=I65  Ipu=off  Pbase=100e6  Vbase=24900  OutputType=Complex  PhasorSimulation=on  PSBequivalent=0
      settings: SourceProductName=Simscape Electrical
  62 Y Z : powerlib/Elements/Series RLC Load  LConnTagsString=a  RConnTagsString=__new0  NominalVoltage=1.0*2401.78  NominalFrequency=60  ActivePower=40e3*a  InductivePower=20e3*a  CapacitivePower=0  Setx0=off  InitialVoltage=0  SetiL0=off  InitialCurrent=0  Measurements=None  LoadType=constant Z
      settings: SourceProductName=Simscape Electrical
  62-63 12 : powerlib/Elements/Three-Phase PI Section Line  LConnTagsString=a|b|c  RConnTagsString=A|B|C  Frequency=60  Resistances=[R1_12 R0_12]  Inductances=[L1_12 L0_12]  Capacitances=[C1_12 C0_12]  Length=175*ft2km
      settings: SourceProductName=Simscape Electrical
  63 : powerlib/Measurements/Three-Phase V-I Measurement  VoltageMeasurement=phase-to-ground  SetLabelV=on  LabelV=V63  Vpu=off  VpuLL=off  CurrentMeasurement=no  SetLabelI=on  LabelI=I65  Ipu=off  Pbase=100e6  Vbase=24900  OutputType=Complex  PhasorSimulation=on  PSBequivalent=0
      settings: SourceProductName=Simscape Electrical
  63 Y PQ : powerlib/Elements/Series RLC Load  LConnTagsString=a  RConnTagsString=__new0  NominalVoltage=1.0*2401.78  NominalFrequency=60  ActivePower=40e3*a  InductivePower=20e3*a  CapacitivePower=0  Setx0=off  InitialVoltage=0  SetiL0=off  InitialCurrent=0  Measurements=None  LoadType=constant PQ
      settings: SourceProductName=Simscape Electrical
  63-64 12 : powerlib/Elements/Three-Phase PI Section Line  LConnTagsString=a|b|c  RConnTagsString=A|B|C  Frequency=60  Resistances=[R1_12 R0_12]  Inductances=[L1_12 L0_12]  Capacitances=[C1_12 C0_12]  Length=350*ft2km
      settings: SourceProductName=Simscape Electrical
  64 : powerlib/Measurements/Three-Phase V-I Measurement  VoltageMeasurement=phase-to-ground  SetLabelV=on  LabelV=V64  Vpu=off  VpuLL=off  CurrentMeasurement=no  SetLabelI=on  LabelI=I65  Ipu=off  Pbase=100e6  Vbase=24900  OutputType=Complex  PhasorSimulation=on  PSBequivalent=0
      settings: SourceProductName=Simscape Electrical
  64 Y I : powerlib/Elements/Series RLC Load  LConnTagsString=a  RConnTagsString=__new0  NominalVoltage=1.0*2401.78  NominalFrequency=60  ActivePower=75e3*a  InductivePower=35e3*a  CapacitivePower=0  Setx0=off  InitialVoltage=0  SetiL0=off  InitialCurrent=0  Measurements=None  LoadType=constant I
      settings: SourceProductName=Simscape Electrical
  64-65 12 : powerlib/Elements/Three-Phase PI Section Line  LConnTagsString=a|b|c  RConnTagsString=A|B|C  Frequency=60  Resistances=[R1_12 R0_12]  Inductances=[L1_12 L0_12]  Capacitances=[C1_12 C0_12]  Length=425*ft2km
      settings: SourceProductName=Simscape Electrical
  65 : powerlib/Measurements/Three-Phase V-I Measurement  VoltageMeasurement=phase-to-ground  SetLabelV=on  LabelV=V65  Vpu=off  VpuLL=off  CurrentMeasurement=yes  SetLabelI=on  LabelI=I65  Ipu=off  Pbase=100e6  Vbase=24900  OutputType=Complex  PhasorSimulation=on  PSBequivalent=0
      settings: SourceProductName=Simscape Electrical
  65 D Z : powerlib/Elements/Three-Phase Series RLC Load  LConnTagsString=A|B|C  Configuration=Delta  NominalVoltage=120e3  Vabc=[ 1.0 1.0 1.0]*2401.78  Vabcp=[ 1.0 1.0 1.0]*4160  NominalFrequency=60  UnbalancedPower=on  ActivePower=1e+006  InductivePower=0  CapacitivePower=0  Pabc="[17 66  117]*1e3/2"  QLabc="[10 38  68]*1e3/2"  QCabc=[0 0 0]  Pabcp=[35 35 70]*1e3*a  QLabcp=[25 25 50]*1e3*a  QCabcp=[0 0 0]  Measurements=None  LoadType=constant Z
      settings: SourceProductName=Simscape Electrical
  65-66 12 : powerlib/Elements/Three-Phase PI Section Line  LConnTagsString=a|b|c  RConnTagsString=A|B|C  Frequency=60  Resistances=[R1_12 R0_12]  Inductances=[L1_12 L0_12]  Capacitances=[C1_12 C0_12]  Length=325*ft2km
      settings: SourceProductName=Simscape Electrical
  66 : powerlib/Measurements/Three-Phase V-I Measurement  VoltageMeasurement=phase-to-ground  SetLabelV=on  LabelV=V66  Vpu=off  VpuLL=off  CurrentMeasurement=no  SetLabelI=on  LabelI=I65  Ipu=off  Pbase=100e6  Vbase=24900  OutputType=Complex  PhasorSimulation=on  PSBequivalent=0
      settings: SourceProductName=Simscape Electrical
  66 Y PQ : powerlib/Elements/Series RLC Load  LConnTagsString=a  RConnTagsString=__new0  NominalVoltage=1.0*2401.78  NominalFrequency=60  ActivePower=75e3*a  InductivePower=35e3*a  CapacitivePower=0  Setx0=off  InitialVoltage=0  SetiL0=off  InitialCurrent=0  Measurements=None  LoadType=constant PQ
      settings: SourceProductName=Simscape Electrical
  67 : powerlib/Measurements/Three-Phase V-I Measurement  VoltageMeasurement=phase-to-ground  SetLabelV=on  LabelV=V67  Vpu=off  VpuLL=off  CurrentMeasurement=no  SetLabelI=on  LabelI=I65  Ipu=off  Pbase=100e6  Vbase=24900  OutputType=Complex  PhasorSimulation=on  PSBequivalent=0
      settings: SourceProductName=Simscape Electrical
  67-68 9 : powerlib/Elements/Pi Section Line  LConnTagsString=__new0  RConnTagsString=__new0  Frequency=60  Resistance=R1_9  Inductance=L1_9  Capacitance=C1_9  Length=200*ft2km  PiSections=1  Measurements=None
      settings: AttributesFormatString=\n  SourceProductName=Simscape Electrical  SourceProductBaseCode=PS
  67-72 3 : powerlib/Elements/Three-Phase PI Section Line  LConnTagsString=a|b|c  RConnTagsString=A|B|C  Frequency=60  Resistances=[R1_3 R0_3]  Inductances=[L1_3 L0_3]  Capacitances=[C1_3 C0_3]  Length=275*ft2km
      settings: SourceProductName=Simscape Electrical
  67-97 3 : Subsystem  mask(Three-Phase PI Section Block){Rl=R_3, Ll=L_3, Cl=C_3, L=350*ft2km}
      mask prompts: Rl "Resistance per unit Length(Ohm/Km)[3x3 matrix]"; Ll "Inductance per unit Length(H/Km)[3x3 matrix]"; Cl "Capacitance per unit Length(F/Km)[3x3 matrix]"; L "Length (Km)"
      mask help: This block models a three-phase transmission line with a single PI section.
  68 : Subsystem
  68 Y PQ : powerlib/Elements/Series RLC Load  LConnTagsString=a  RConnTagsString=__new0  NominalVoltage=1.0*2401.78  NominalFrequency=60  ActivePower=20e3*a  InductivePower=10e3*a  CapacitivePower=0  Setx0=off  InitialVoltage=0  SetiL0=off  InitialCurrent=0  Measurements=None  LoadType=constant PQ
      settings: SourceProductName=Simscape Electrical
  68-69 9 : powerlib/Elements/Pi Section Line  LConnTagsString=__new0  RConnTagsString=__new0  Frequency=60  Resistance=R1_9  Inductance=L1_9  Capacitance=C1_9  Length=275*ft2km  PiSections=1  Measurements=None
      settings: AttributesFormatString=\n  SourceProductName=Simscape Electrical  SourceProductBaseCode=PS
  69 : Subsystem
  69 Y PQ : powerlib/Elements/Series RLC Load  LConnTagsString=a  RConnTagsString=__new0  NominalVoltage=1.0*2401.78  NominalFrequency=60  ActivePower=40e3*a  InductivePower=20e3*a  CapacitivePower=0  Setx0=off  InitialVoltage=0  SetiL0=off  InitialCurrent=0  Measurements=None  LoadType=constant PQ
      settings: SourceProductName=Simscape Electrical
  69-70 9 : powerlib/Elements/Pi Section Line  LConnTagsString=__new0  RConnTagsString=__new0  Frequency=60  Resistance=R1_9  Inductance=L1_9  Capacitance=C1_9  Length=325*ft2km  PiSections=1  Measurements=None
      settings: AttributesFormatString=\n  SourceProductName=Simscape Electrical  SourceProductBaseCode=PS
  7 : powerlib/Measurements/Three-Phase V-I Measurement  VoltageMeasurement=phase-to-ground  SetLabelV=on  LabelV=V7  Vpu=off  VpuLL=off  CurrentMeasurement=no  SetLabelI=on  LabelI=I800  Ipu=off  Pbase=100e6  Vbase=24900  OutputType=Complex  PhasorSimulation=on  PSBequivalent=0
      settings: SourceProductName=Simscape Electrical
  7 Y PQ : powerlib/Elements/Series RLC Load  LConnTagsString=a  RConnTagsString=__new0  NominalVoltage=1.0*2401.78  NominalFrequency=60  ActivePower=20e3*a  InductivePower=10e3*a  CapacitivePower=0  Setx0=off  InitialVoltage=0  SetiL0=off  InitialCurrent=0  Measurements=None  LoadType=constant PQ
      settings: SourceProductName=Simscape Electrical
  7-8 1 : powerlib/Elements/Three-Phase PI Section Line  LConnTagsString=a|b|c  RConnTagsString=A|B|C  Frequency=60  Resistances=[R1_1 R0_1]  Inductances=[L1_1 L0_1]  Capacitances=[C1_1 C0_1]  Length=200*ft2km
      settings: SourceProductName=Simscape Electrical
  70 : Subsystem
  70 Y PQ : powerlib/Elements/Series RLC Load  LConnTagsString=a  RConnTagsString=__new0  NominalVoltage=1.0*2401.78  NominalFrequency=60  ActivePower=20e3*a  InductivePower=10e3*a  CapacitivePower=0  Setx0=off  InitialVoltage=0  SetiL0=off  InitialCurrent=0  Measurements=None  LoadType=constant PQ
      settings: SourceProductName=Simscape Electrical
  70-71 1 : powerlib/Elements/Pi Section Line  LConnTagsString=__new0  RConnTagsString=__new0  Frequency=60  Resistance=R1_9  Inductance=L1_9  Capacitance=C1_9  Length=275*ft2km  PiSections=1  Measurements=None
      settings: AttributesFormatString=\n  SourceProductName=Simscape Electrical  SourceProductBaseCode=PS
  71 : Subsystem
  71 Y PQ : powerlib/Elements/Series RLC Load  LConnTagsString=a  RConnTagsString=__new0  NominalVoltage=1.0*2401.78  NominalFrequency=60  ActivePower=40e3*a  InductivePower=20e3*a  CapacitivePower=0  Setx0=off  InitialVoltage=0  SetiL0=off  InitialCurrent=0  Measurements=None  LoadType=constant PQ
      settings: SourceProductName=Simscape Electrical
  72 : powerlib/Measurements/Three-Phase V-I Measurement  VoltageMeasurement=phase-to-ground  SetLabelV=on  LabelV=V72  Vpu=off  VpuLL=off  CurrentMeasurement=no  SetLabelI=on  LabelI=I65  Ipu=off  Pbase=100e6  Vbase=24900  OutputType=Complex  PhasorSimulation=on  PSBequivalent=0
      settings: SourceProductName=Simscape Electrical
  72-73 11 : powerlib/Elements/Pi Section Line  LConnTagsString=__new0  RConnTagsString=__new0  Frequency=60  Resistance=R1_11  Inductance=L1_11  Capacitance=C1_11  Length=275*ft2km  PiSections=1  Measurements=None
      settings: AttributesFormatString=\n  SourceProductName=Simscape Electrical  SourceProductBaseCode=PS
  72-76 3 : powerlib/Elements/Three-Phase PI Section Line  LConnTagsString=a|b|c  RConnTagsString=A|B|C  Frequency=60  Resistances=[R1_3 R0_3]  Inductances=[L1_3 L0_3]  Capacitances=[C1_3 C0_3]  Length=200*ft2km
      settings: SourceProductName=Simscape Electrical
  73 : Subsystem
  73 Y PQ : powerlib/Elements/Series RLC Load  LConnTagsString=a  RConnTagsString=__new0  NominalVoltage=1.0*2401.78  NominalFrequency=60  ActivePower=40e3*a  InductivePower=20e3*a  CapacitivePower=0  Setx0=off  InitialVoltage=0  SetiL0=off  InitialCurrent=0  Measurements=None  LoadType=constant PQ
      settings: SourceProductName=Simscape Electrical
  73-74 11 : powerlib/Elements/Pi Section Line  LConnTagsString=__new0  RConnTagsString=__new0  Frequency=60  Resistance=R1_11  Inductance=L1_11  Capacitance=C1_11  Length=350*ft2km  PiSections=1  Measurements=None
      settings: AttributesFormatString=\n  SourceProductName=Simscape Electrical  SourceProductBaseCode=PS
  74 : Subsystem
  74 Y Z : powerlib/Elements/Series RLC Load  LConnTagsString=a  RConnTagsString=__new0  NominalVoltage=1.0*2401.78  NominalFrequency=60  ActivePower=40e3*a  InductivePower=20e3*a  CapacitivePower=0  Setx0=off  InitialVoltage=0  SetiL0=off  InitialCurrent=0  Measurements=None  LoadType=constant Z
      settings: SourceProductName=Simscape Electrical
  74-75 11 : powerlib/Elements/Pi Section Line  LConnTagsString=__new0  RConnTagsString=__new0  Frequency=60  Resistance=R1_11  Inductance=L1_11  Capacitance=C1_11  Length=400*ft2km  PiSections=1  Measurements=None
      settings: AttributesFormatString=\n  SourceProductName=Simscape Electrical  SourceProductBaseCode=PS
  75 : Subsystem
  75 Y PQ : powerlib/Elements/Series RLC Load  LConnTagsString=a  RConnTagsString=__new0  NominalVoltage=1.0*2401.78  NominalFrequency=60  ActivePower=40e3*a  InductivePower=20e3*a  CapacitivePower=0  Setx0=off  InitialVoltage=0  SetiL0=off  InitialCurrent=0  Measurements=None  LoadType=constant PQ
      settings: SourceProductName=Simscape Electrical
  76 : powerlib/Measurements/Three-Phase V-I Measurement  VoltageMeasurement=phase-to-ground  SetLabelV=on  LabelV=V76  Vpu=off  VpuLL=off  CurrentMeasurement=no  SetLabelI=on  LabelI=I65  Ipu=off  Pbase=100e6  Vbase=24900  OutputType=Complex  PhasorSimulation=on  PSBequivalent=0
      settings: SourceProductName=Simscape Electrical
  76 DI : powerlib/Elements/Three-Phase Series RLC Load  LConnTagsString=A|B|C  Configuration=Delta  NominalVoltage=120e3  Vabc=[ 1.0 1.0 1.0]*2401.78  Vabcp=[ 1.0 1.0 1.0]*4160  NominalFrequency=60  UnbalancedPower=on  ActivePower=1e+006  InductivePower=0  CapacitivePower=0  Pabc="[17 66  117]*1e3/2"  QLabc="[10 38  68]*1e3/2"  QCabc=[0 0 0]  Pabcp="[105 70  70]*1e3*a"  QLabcp=[80 50 50]*1e3*a  QCabcp=[0 0 0]  Measurements=None  LoadType=constant I
      settings: SourceProductName=Simscape Electrical
  76-77 6 : powerlib/Elements/Three-Phase PI Section Line  LConnTagsString=a|b|c  RConnTagsString=A|B|C  Frequency=60  Resistances=[R1_6 R0_6]  Inductances=[L1_6 L0_6]  Capacitances=[C1_6 C0_6]  Length=400*ft2km
      settings: SourceProductName=Simscape Electrical
  76-86 3 : powerlib/Elements/Three-Phase PI Section Line  LConnTagsString=a|b|c  RConnTagsString=A|B|C  Frequency=60  Resistances=[R1_3 R0_3]  Inductances=[L1_3 L0_3]  Capacitances=[C1_3 C0_3]  Length=700*ft2km
      settings: SourceProductName=Simscape Electrical
  77 : powerlib/Measurements/Three-Phase V-I Measurement  VoltageMeasurement=phase-to-ground  SetLabelV=on  LabelV=V77  Vpu=off  VpuLL=off  CurrentMeasurement=no  SetLabelI=on  LabelI=I65  Ipu=off  Pbase=100e6  Vbase=24900  OutputType=Complex  PhasorSimulation=on  PSBequivalent=0
      settings: SourceProductName=Simscape Electrical
  77 Y PQ : powerlib/Elements/Series RLC Load  LConnTagsString=a  RConnTagsString=__new0  NominalVoltage=1.0*2401.78  NominalFrequency=60  ActivePower=40e3*a  InductivePower=20e3*a  CapacitivePower=0  Setx0=off  InitialVoltage=0  SetiL0=off  InitialCurrent=0  Measurements=None  LoadType=constant PQ
      settings: SourceProductName=Simscape Electrical
  77-78 6 : powerlib/Elements/Three-Phase PI Section Line  LConnTagsString=a|b|c  RConnTagsString=A|B|C  Frequency=60  Resistances=[R1_6 R0_6]  Inductances=[L1_6 L0_6]  Capacitances=[C1_6 C0_6]  Length=100*ft2km
      settings: SourceProductName=Simscape Electrical
  78 : powerlib/Measurements/Three-Phase V-I Measurement  VoltageMeasurement=phase-to-ground  SetLabelV=on  LabelV=V78  Vpu=off  VpuLL=off  CurrentMeasurement=no  SetLabelI=on  LabelI=I65  Ipu=off  Pbase=100e6  Vbase=24900  OutputType=Complex  PhasorSimulation=on  PSBequivalent=0
      settings: SourceProductName=Simscape Electrical
  78-79 6 : powerlib/Elements/Three-Phase PI Section Line  LConnTagsString=a|b|c  RConnTagsString=A|B|C  Frequency=60  Resistances=[R1_6 R0_6]  Inductances=[L1_6 L0_6]  Capacitances=[C1_6 C0_6]  Length=225*ft2km
      settings: SourceProductName=Simscape Electrical
  78-80 6 : powerlib/Elements/Three-Phase PI Section Line  LConnTagsString=a|b|c  RConnTagsString=A|B|C  Frequency=60  Resistances=[R1_6 R0_6]  Inductances=[L1_6 L0_6]  Capacitances=[C1_6 C0_6]  Length=475*ft2km
      settings: SourceProductName=Simscape Electrical
  79 : powerlib/Measurements/Three-Phase V-I Measurement  VoltageMeasurement=phase-to-ground  SetLabelV=on  LabelV=V79  Vpu=off  VpuLL=off  CurrentMeasurement=no  SetLabelI=on  LabelI=I65  Ipu=off  Pbase=100e6  Vbase=24900  OutputType=Complex  PhasorSimulation=on  PSBequivalent=0
      settings: SourceProductName=Simscape Electrical
  79 Y Z : powerlib/Elements/Series RLC Load  LConnTagsString=a  RConnTagsString=__new0  NominalVoltage=1.0*2401.78  NominalFrequency=60  ActivePower=40e3*a  InductivePower=20e3*a  CapacitivePower=0  Setx0=off  InitialVoltage=0  SetiL0=off  InitialCurrent=0  Measurements=None  LoadType=constant Z
      settings: SourceProductName=Simscape Electrical
  8 : powerlib/Measurements/Three-Phase V-I Measurement  VoltageMeasurement=phase-to-ground  SetLabelV=on  LabelV=V8  Vpu=off  VpuLL=off  CurrentMeasurement=no  SetLabelI=on  LabelI=I800  Ipu=off  Pbase=100e6  Vbase=24900  OutputType=Complex  PhasorSimulation=on  PSBequivalent=0
      settings: SourceProductName=Simscape Electrical
  8-12 10 : powerlib/Elements/Pi Section Line  LConnTagsString=__new0  RConnTagsString=__new0  Frequency=60  Resistance=R1_10  Inductance=L1_10  Capacitance=C1_10  Length=225*ft2km  PiSections=1  Measurements=None
      settings: AttributesFormatString=\n  SourceProductName=Simscape Electrical  SourceProductBaseCode=PS
  8-13 1 : powerlib/Elements/Three-Phase PI Section Line  LConnTagsString=a|b|c  RConnTagsString=A|B|C  Frequency=60  Resistances=[R1_1 R0_1]  Inductances=[L1_1 L0_1]  Capacitances=[C1_1 C0_1]  Length=300*ft2km
      settings: SourceProductName=Simscape Electrical
  8-9 9 : powerlib/Elements/Pi Section Line  LConnTagsString=__new0  RConnTagsString=__new0  Frequency=60  Resistance=R1_9  Inductance=L1_9  Capacitance=C1_9  Length=225*ft2km  PiSections=1  Measurements=None
      settings: AttributesFormatString=\n  SourceProductName=Simscape Electrical  SourceProductBaseCode=PS
  80 : powerlib/Measurements/Three-Phase V-I Measurement  VoltageMeasurement=phase-to-ground  SetLabelV=on  LabelV=V80  Vpu=off  VpuLL=off  CurrentMeasurement=no  SetLabelI=on  LabelI=I65  Ipu=off  Pbase=100e6  Vbase=24900  OutputType=Complex  PhasorSimulation=on  PSBequivalent=0
      settings: SourceProductName=Simscape Electrical
  80 Y PQ : powerlib/Elements/Series RLC Load  LConnTagsString=a  RConnTagsString=__new0  NominalVoltage=1.0*2401.78  NominalFrequency=60  ActivePower=40e3*a  InductivePower=20e3*a  CapacitivePower=0  Setx0=off  InitialVoltage=0  SetiL0=off  InitialCurrent=0  Measurements=None  LoadType=constant PQ
      settings: SourceProductName=Simscape Electrical
  80-81 6 : powerlib/Elements/Three-Phase PI Section Line  LConnTagsString=a|b|c  RConnTagsString=A|B|C  Frequency=60  Resistances=[R1_6 R0_6]  Inductances=[L1_6 L0_6]  Capacitances=[C1_6 C0_6]  Length=475*ft2km
      settings: SourceProductName=Simscape Electrical
  81 : powerlib/Measurements/Three-Phase V-I Measurement  VoltageMeasurement=phase-to-ground  SetLabelV=on  LabelV=V81  Vpu=off  VpuLL=off  CurrentMeasurement=no  SetLabelI=on  LabelI=I65  Ipu=off  Pbase=100e6  Vbase=24900  OutputType=Complex  PhasorSimulation=on  PSBequivalent=0
      settings: SourceProductName=Simscape Electrical
  81-82 6 : powerlib/Elements/Three-Phase PI Section Line  LConnTagsString=a|b|c  RConnTagsString=A|B|C  Frequency=60  Resistances=[R1_6 R0_6]  Inductances=[L1_6 L0_6]  Capacitances=[C1_6 C0_6]  Length=250*ft2km
      settings: SourceProductName=Simscape Electrical
  81-84 11 : powerlib/Elements/Pi Section Line  LConnTagsString=__new0  RConnTagsString=__new0  Frequency=60  Resistance=R1_11  Inductance=L1_11  Capacitance=C1_11  Length=675*ft2km  PiSections=1  Measurements=None
      settings: AttributesFormatString=\n  SourceProductName=Simscape Electrical  SourceProductBaseCode=PS
  82 : powerlib/Measurements/Three-Phase V-I Measurement  VoltageMeasurement=phase-to-ground  SetLabelV=on  LabelV=V82  Vpu=off  VpuLL=off  CurrentMeasurement=no  SetLabelI=on  LabelI=I65  Ipu=off  Pbase=100e6  Vbase=24900  OutputType=Complex  PhasorSimulation=on  PSBequivalent=0
      settings: SourceProductName=Simscape Electrical
  82 Y PQ : powerlib/Elements/Series RLC Load  LConnTagsString=a  RConnTagsString=__new0  NominalVoltage=1.0*2401.78  NominalFrequency=60  ActivePower=40e3*a  InductivePower=20e3*a  CapacitivePower=0  Setx0=off  InitialVoltage=0  SetiL0=off  InitialCurrent=0  Measurements=None  LoadType=constant PQ
      settings: SourceProductName=Simscape Electrical
  82-83 6 : powerlib/Elements/Three-Phase PI Section Line  LConnTagsString=a|b|c  RConnTagsString=A|B|C  Frequency=60  Resistances=[R1_6 R0_6]  Inductances=[L1_6 L0_6]  Capacitances=[C1_6 C0_6]  Length=250*ft2km
      settings: SourceProductName=Simscape Electrical
  83 : powerlib/Measurements/Three-Phase V-I Measurement  VoltageMeasurement=phase-to-ground  SetLabelV=on  LabelV=V83  Vpu=off  VpuLL=off  CurrentMeasurement=no  SetLabelI=on  LabelI=I65  Ipu=off  Pbase=100e6  Vbase=24900  OutputType=Complex  PhasorSimulation=on  PSBequivalent=0
      settings: SourceProductName=Simscape Electrical
  83 Y CAP : powerlib/Elements/Three-Phase Series RLC Load  LConnTagsString=A|B|C  Configuration=Y (grounded)  NominalVoltage=120e3  Vabc=[ 1.0 1.0 1.0]*2401.78  Vabcp=[1e3 1e3 1e3]  NominalFrequency=60  UnbalancedPower=on  ActivePower=1e+006  InductivePower=0  CapacitivePower=0  Pabc=[0 0 0 ]*1e3  QLabc=[0 0 0 ]*1e3  QCabc=[200 200 200]*1e3*a  Pabcp=[10e3 9e3 11e3]  QLabcp=[100 90 110]  QCabcp=[100 90 110]  Measurements=None  LoadType=constant Z
      settings: SourceProductName=Simscape Electrical
  83 Y PQ : powerlib/Elements/Series RLC Load  LConnTagsString=a  RConnTagsString=__new0  NominalVoltage=1.0*2401.78  NominalFrequency=60  ActivePower=20e3*a  InductivePower=10e3*a  CapacitivePower=0  Setx0=off  InitialVoltage=0  SetiL0=off  InitialCurrent=0  Measurements=None  LoadType=constant PQ
      settings: SourceProductName=Simscape Electrical
  84 : Subsystem
  84 Y PQ : powerlib/Elements/Series RLC Load  LConnTagsString=a  RConnTagsString=__new0  NominalVoltage=1.0*2401.78  NominalFrequency=60  ActivePower=20e3*a  InductivePower=10e3*a  CapacitivePower=0  Setx0=off  InitialVoltage=0  SetiL0=off  InitialCurrent=0  Measurements=None  LoadType=constant PQ
      settings: SourceProductName=Simscape Electrical
  84-85 11 : powerlib/Elements/Pi Section Line  LConnTagsString=__new0  RConnTagsString=__new0  Frequency=60  Resistance=R1_11  Inductance=L1_11  Capacitance=C1_11  Length=475*ft2km  PiSections=1  Measurements=None
      settings: AttributesFormatString=\n  SourceProductName=Simscape Electrical  SourceProductBaseCode=PS
  85 : Subsystem
  85 Y PQ : powerlib/Elements/Series RLC Load  LConnTagsString=a  RConnTagsString=__new0  NominalVoltage=1.0*2401.78  NominalFrequency=60  ActivePower=40e3*a  InductivePower=20e3*a  CapacitivePower=0  Setx0=off  InitialVoltage=0  SetiL0=off  InitialCurrent=0  Measurements=None  LoadType=constant PQ
      settings: SourceProductName=Simscape Electrical
  86 : powerlib/Measurements/Three-Phase V-I Measurement  VoltageMeasurement=phase-to-ground  SetLabelV=on  LabelV=V86  Vpu=off  VpuLL=off  CurrentMeasurement=no  SetLabelI=on  LabelI=I65  Ipu=off  Pbase=100e6  Vbase=24900  OutputType=Complex  PhasorSimulation=on  PSBequivalent=0
      settings: SourceProductName=Simscape Electrical
  86 Y PQ : powerlib/Elements/Series RLC Load  LConnTagsString=a  RConnTagsString=__new0  NominalVoltage=1.0*2401.78  NominalFrequency=60  ActivePower=20e3*a  InductivePower=10e3*a  CapacitivePower=0  Setx0=off  InitialVoltage=0  SetiL0=off  InitialCurrent=0  Measurements=None  LoadType=constant PQ
      settings: SourceProductName=Simscape Electrical
  86-87 6 : powerlib/Elements/Three-Phase PI Section Line  LConnTagsString=a|b|c  RConnTagsString=A|B|C  Frequency=60  Resistances=[R1_6 R0_6]  Inductances=[L1_6 L0_6]  Capacitances=[C1_6 C0_6]  Length=450*ft2km
      settings: SourceProductName=Simscape Electrical
  87 : powerlib/Measurements/Three-Phase V-I Measurement  VoltageMeasurement=phase-to-ground  SetLabelV=on  LabelV=V87  Vpu=off  VpuLL=off  CurrentMeasurement=no  SetLabelI=on  LabelI=I65  Ipu=off  Pbase=100e6  Vbase=24900  OutputType=Complex  PhasorSimulation=on  PSBequivalent=0
      settings: SourceProductName=Simscape Electrical
  87 Y PQ : powerlib/Elements/Series RLC Load  LConnTagsString=a  RConnTagsString=__new0  NominalVoltage=1.0*2401.78  NominalFrequency=60  ActivePower=40e3*a  InductivePower=20e3*a  CapacitivePower=0  Setx0=off  InitialVoltage=0  SetiL0=off  InitialCurrent=0  Measurements=None  LoadType=constant PQ
      settings: SourceProductName=Simscape Electrical
  87-88 9 : powerlib/Elements/Pi Section Line  LConnTagsString=__new0  RConnTagsString=__new0  Frequency=60  Resistance=R1_9  Inductance=L1_9  Capacitance=C1_9  Length=175*ft2km  PiSections=1  Measurements=None
      settings: AttributesFormatString=\n  SourceProductName=Simscape Electrical  SourceProductBaseCode=PS
  87-89 6 : powerlib/Elements/Three-Phase PI Section Line  LConnTagsString=a|b|c  RConnTagsString=A|B|C  Frequency=60  Resistances=[R1_6 R0_6]  Inductances=[L1_6 L0_6]  Capacitances=[C1_6 C0_6]  Length=250*ft2km
      settings: SourceProductName=Simscape Electrical
  88 : Subsystem
  88 Y CAP : powerlib/Elements/Series RLC Load  LConnTagsString=a  RConnTagsString=__new0  NominalVoltage=1.0*2401.78  NominalFrequency=60  ActivePower=0  InductivePower=0  CapacitivePower=50e3*a  Setx0=off  InitialVoltage=0  SetiL0=off  InitialCurrent=0  Measurements=None  LoadType=constant PQ
      settings: SourceProductName=Simscape Electrical
  88 Y PQ : powerlib/Elements/Series RLC Load  LConnTagsString=a  RConnTagsString=__new0  NominalVoltage=1.0*2401.78  NominalFrequency=60  ActivePower=40e3*a  InductivePower=20e3*a  CapacitivePower=0  Setx0=off  InitialVoltage=0  SetiL0=off  InitialCurrent=0  Measurements=None  LoadType=constant PQ
      settings: SourceProductName=Simscape Electrical
  89 : powerlib/Measurements/Three-Phase V-I Measurement  VoltageMeasurement=phase-to-ground  SetLabelV=on  LabelV=V89  Vpu=off  VpuLL=off  CurrentMeasurement=no  SetLabelI=on  LabelI=I65  Ipu=off  Pbase=100e6  Vbase=24900  OutputType=Complex  PhasorSimulation=on  PSBequivalent=0
      settings: SourceProductName=Simscape Electrical
  89-90 10 : powerlib/Elements/Pi Section Line  LConnTagsString=__new0  RConnTagsString=__new0  Frequency=60  Resistance=R1_10  Inductance=L1_10  Capacitance=C1_10  Length=225*ft2km  PiSections=1  Measurements=None
      settings: AttributesFormatString=\n  SourceProductName=Simscape Electrical  SourceProductBaseCode=PS
  89-91 6 : powerlib/Elements/Three-Phase PI Section Line  LConnTagsString=a|b|c  RConnTagsString=A|B|C  Frequency=60  Resistances=[R1_6 R0_6]  Inductances=[L1_6 L0_6]  Capacitances=[C1_6 C0_6]  Length=225*ft2km
      settings: SourceProductName=Simscape Electrical
  9 : Subsystem
  9 Y PQ : powerlib/Elements/Series RLC Load  LConnTagsString=a  RConnTagsString=__new0  NominalVoltage=1.0*2401.78  NominalFrequency=60  ActivePower=40e3*a  InductivePower=20e3*a  CapacitivePower=0  Setx0=off  InitialVoltage=0  SetiL0=off  InitialCurrent=0  Measurements=None  LoadType=constant PQ
      settings: SourceProductName=Simscape Electrical
  9-14 9 : powerlib/Elements/Pi Section Line  LConnTagsString=__new0  RConnTagsString=__new0  Frequency=60  Resistance=R1_9  Inductance=L1_9  Capacitance=C1_9  Length=425*ft2km  PiSections=1  Measurements=None
      settings: AttributesFormatString=\n  SourceProductName=Simscape Electrical  SourceProductBaseCode=PS
  90 : Subsystem
  90 Y CAP : powerlib/Elements/Series RLC Load  LConnTagsString=a  RConnTagsString=__new0  NominalVoltage=1.0*2401.78  NominalFrequency=60  ActivePower=0  InductivePower=0  CapacitivePower=50e3*a  Setx0=off  InitialVoltage=0  SetiL0=off  InitialCurrent=0  Measurements=None  LoadType=constant PQ
      settings: SourceProductName=Simscape Electrical
  90 Y I : powerlib/Elements/Series RLC Load  LConnTagsString=a  RConnTagsString=__new0  NominalVoltage=1.0*2401.78  NominalFrequency=60  ActivePower=40e3*a  InductivePower=20e3*a  CapacitivePower=0  Setx0=off  InitialVoltage=0  SetiL0=off  InitialCurrent=0  Measurements=None  LoadType=constant I
      settings: SourceProductName=Simscape Electrical
  91 : powerlib/Measurements/Three-Phase V-I Measurement  VoltageMeasurement=phase-to-ground  SetLabelV=on  LabelV=V91  Vpu=off  VpuLL=off  CurrentMeasurement=no  SetLabelI=on  LabelI=I65  Ipu=off  Pbase=100e6  Vbase=24900  OutputType=Complex  PhasorSimulation=on  PSBequivalent=0
      settings: SourceProductName=Simscape Electrical
  91-92 11 : powerlib/Elements/Pi Section Line  LConnTagsString=__new0  RConnTagsString=__new0  Frequency=60  Resistance=R1_11  Inductance=L1_11  Capacitance=C1_11  Length=300*ft2km  PiSections=1  Measurements=None
      settings: AttributesFormatString=\n  SourceProductName=Simscape Electrical  SourceProductBaseCode=PS
  91-93 6 : powerlib/Elements/Three-Phase PI Section Line  LConnTagsString=a|b|c  RConnTagsString=A|B|C  Frequency=60  Resistances=[R1_6 R0_6]  Inductances=[L1_6 L0_6]  Capacitances=[C1_6 C0_6]  Length=225*ft2km
      settings: SourceProductName=Simscape Electrical
  92 : Subsystem
  92 Y CAP : powerlib/Elements/Series RLC Load  LConnTagsString=a  RConnTagsString=__new0  NominalVoltage=1.0*2401.78  NominalFrequency=60  ActivePower=0  InductivePower=0  CapacitivePower=50e3*a  Setx0=off  InitialVoltage=0  SetiL0=off  InitialCurrent=0  Measurements=None  LoadType=constant PQ
      settings: SourceProductName=Simscape Electrical
  92 Y PQ : powerlib/Elements/Series RLC Load  LConnTagsString=a  RConnTagsString=__new0  NominalVoltage=1.0*2401.78  NominalFrequency=60  ActivePower=40e3*a  InductivePower=20e3*a  CapacitivePower=0  Setx0=off  InitialVoltage=0  SetiL0=off  InitialCurrent=0  Measurements=None  LoadType=constant PQ
      settings: SourceProductName=Simscape Electrical
  93 : powerlib/Measurements/Three-Phase V-I Measurement  VoltageMeasurement=phase-to-ground  SetLabelV=on  LabelV=V93  Vpu=off  VpuLL=off  CurrentMeasurement=no  SetLabelI=on  LabelI=I65  Ipu=off  Pbase=100e6  Vbase=24900  OutputType=Complex  PhasorSimulation=on  PSBequivalent=0
      settings: SourceProductName=Simscape Electrical
  93-94 9 : powerlib/Elements/Pi Section Line  LConnTagsString=__new0  RConnTagsString=__new0  Frequency=60  Resistance=R1_9  Inductance=L1_9  Capacitance=C1_9  Length=275*ft2km  PiSections=1  Measurements=None
      settings: AttributesFormatString=\n  SourceProductName=Simscape Electrical  SourceProductBaseCode=PS
  93-95 6 : powerlib/Elements/Three-Phase PI Section Line  LConnTagsString=a|b|c  RConnTagsString=A|B|C  Frequency=60  Resistances=[R1_6 R0_6]  Inductances=[L1_6 L0_6]  Capacitances=[C1_6 C0_6]  Length=300*ft2km
      settings: SourceProductName=Simscape Electrical
  94 : Subsystem
  94 Y PQ : powerlib/Elements/Series RLC Load  LConnTagsString=a  RConnTagsString=__new0  NominalVoltage=1.0*2401.78  NominalFrequency=60  ActivePower=40e3*a  InductivePower=20e3*a  CapacitivePower=0  Setx0=off  InitialVoltage=0  SetiL0=off  InitialCurrent=0  Measurements=None  LoadType=constant PQ
      settings: SourceProductName=Simscape Electrical
  95 : powerlib/Measurements/Three-Phase V-I Measurement  VoltageMeasurement=phase-to-ground  SetLabelV=on  LabelV=V95  Vpu=off  VpuLL=off  CurrentMeasurement=no  SetLabelI=on  LabelI=I65  Ipu=off  Pbase=100e6  Vbase=24900  OutputType=Complex  PhasorSimulation=on  PSBequivalent=0
      settings: SourceProductName=Simscape Electrical
  95 Y PQ : powerlib/Elements/Series RLC Load  LConnTagsString=a  RConnTagsString=__new0  NominalVoltage=1.0*2401.78  NominalFrequency=60  ActivePower=20e3*a  InductivePower=10e3*a  CapacitivePower=0  Setx0=off  InitialVoltage=0  SetiL0=off  InitialCurrent=0  Measurements=None  LoadType=constant PQ
      settings: SourceProductName=Simscape Electrical
  95-96 10 : powerlib/Elements/Pi Section Line  LConnTagsString=__new0  RConnTagsString=__new0  Frequency=60  Resistance=R1_10  Inductance=L1_10  Capacitance=C1_10  Length=200*ft2km  PiSections=1  Measurements=None
      settings: AttributesFormatString=\n  SourceProductName=Simscape Electrical  SourceProductBaseCode=PS
  96 : Subsystem
  96 Y PQ : powerlib/Elements/Series RLC Load  LConnTagsString=a  RConnTagsString=__new0  NominalVoltage=1.0*2401.78  NominalFrequency=60  ActivePower=20e3*a  InductivePower=10e3*a  CapacitivePower=0  Setx0=off  InitialVoltage=0  SetiL0=off  InitialCurrent=0  Measurements=None  LoadType=constant PQ
      settings: SourceProductName=Simscape Electrical
  97 : powerlib/Measurements/Three-Phase V-I Measurement  VoltageMeasurement=phase-to-ground  SetLabelV=on  LabelV=V97  Vpu=off  VpuLL=off  CurrentMeasurement=no  SetLabelI=on  LabelI=I65  Ipu=off  Pbase=100e6  Vbase=24900  OutputType=Complex  PhasorSimulation=on  PSBequivalent=0
      settings: SourceProductName=Simscape Electrical
  97-1 : powerlib/Elements/Three-Phase Breaker  InitialState=closed  SwitchA=off  SwitchB=off  SwitchC=off  SwitchTimes="[1/60  5/60]"  External=off  BreakerResistance=0.01  SnubberResistance=1e6  SnubberCapacitance=inf  Measurements=None
      settings: SourceProductName=Simscape Electrical
  97-98 3 : powerlib/Elements/Three-Phase PI Section Line  LConnTagsString=a|b|c  RConnTagsString=A|B|C  Frequency=60  Resistances=[R1_3 R0_3]  Inductances=[L1_3 L0_3]  Capacitances=[C1_3 C0_3]  Length=275*ft2km
      settings: SourceProductName=Simscape Electrical
  98 : powerlib/Measurements/Three-Phase V-I Measurement  VoltageMeasurement=phase-to-ground  SetLabelV=on  LabelV=V98  Vpu=off  VpuLL=off  CurrentMeasurement=no  SetLabelI=on  LabelI=I65  Ipu=off  Pbase=100e6  Vbase=24900  OutputType=Complex  PhasorSimulation=on  PSBequivalent=0
      settings: SourceProductName=Simscape Electrical
  98 Y PQ : powerlib/Elements/Series RLC Load  LConnTagsString=a  RConnTagsString=__new0  NominalVoltage=1.0*2401.78  NominalFrequency=60  ActivePower=40e3*a  InductivePower=20e3*a  CapacitivePower=0  Setx0=off  InitialVoltage=0  SetiL0=off  InitialCurrent=0  Measurements=None  LoadType=constant PQ
      settings: SourceProductName=Simscape Electrical
  98-99 3 : powerlib/Elements/Three-Phase PI Section Line  LConnTagsString=a|b|c  RConnTagsString=A|B|C  Frequency=60  Resistances=[R1_3 R0_3]  Inductances=[L1_3 L0_3]  Capacitances=[C1_3 C0_3]  Length=550*ft2km
      settings: SourceProductName=Simscape Electrical
  99 : powerlib/Measurements/Three-Phase V-I Measurement  VoltageMeasurement=phase-to-ground  SetLabelV=on  LabelV=V99  Vpu=off  VpuLL=off  CurrentMeasurement=no  SetLabelI=on  LabelI=I65  Ipu=off  Pbase=100e6  Vbase=24900  OutputType=Complex  PhasorSimulation=on  PSBequivalent=0
      settings: SourceProductName=Simscape Electrical
  99 Y PQ : powerlib/Elements/Series RLC Load  LConnTagsString=a  RConnTagsString=__new0  NominalVoltage=1.0*2401.78  NominalFrequency=60  ActivePower=40e3*a  InductivePower=20e3*a  CapacitivePower=0  Setx0=off  InitialVoltage=0  SetiL0=off  InitialCurrent=0  Measurements=None  LoadType=constant PQ
      settings: SourceProductName=Simscape Electrical
  99-100 3 : powerlib/Elements/Three-Phase PI Section Line  LConnTagsString=a|b|c  RConnTagsString=A|B|C  Frequency=60  Resistances=[R1_3 R0_3]  Inductances=[L1_3 L0_3]  Capacitances=[C1_3 C0_3]  Length=300*ft2km
      settings: SourceProductName=Simscape Electrical
  Ground{,1..81} (82 alike) : powerlib/Elements/Ground  LConnTagsString=a
      settings: SourceProductName=Simscape Electrical
  Load Flow Bus1 : powerlib/Measurements/Load Flow Bus  LConnTagsString=a|b  RConnTagsString=a|b  Phases=AC  Connectors=on both sides  ID=27  Vbase=4160/sqrt(3)  Vref=[1.0 1.0]  Vangle=[0 120]  VLF=1  VLFb=1  VLFc=1  angleLF=0  angleLFb=0  angleLFc=0
      settings: SourceProductName=Simscape Electrical
  Load Flow Bus10 : powerlib/Measurements/Load Flow Bus  LConnTagsString=a|b|c  Phases=ABC  Connectors=on one side  ID=251  Vbase=4160/sqrt(3)  Vref=[1.0 1.0 1.0]  Vangle=[0 -120 120]  VLF=1  VLFb=1  VLFc=1  angleLF=0  angleLFb=0  angleLFc=0
      settings: SourceProductName=Simscape Electrical
  Load Flow Bus106 : powerlib/Measurements/Load Flow Bus  LConnTagsString=a|b|c  RConnTagsString=a|b|c  Phases=ABC  Connectors=on both sides  ID=450  Vbase=4160/sqrt(3)  Vref=[1.0 1.0 1.0]  Vangle=[0 -120 120]  VLF=1  VLFb=1  VLFc=1  angleLF=0  angleLFb=0  angleLFc=0
      settings: SourceProductName=Simscape Electrical
  Load Flow Bus107 : powerlib/Measurements/Load Flow Bus  LConnTagsString=a|b|c  Phases=ABC  Connectors=on one side  ID=451  Vbase=4160/sqrt(3)  Vref=[1.0 1.0 1.0]  Vangle=[0 -120 120]  VLF=1  VLFb=1  VLFc=1  angleLF=0  angleLFb=0  angleLFc=0
      settings: SourceProductName=Simscape Electrical
  Load Flow Bus117 : powerlib/Measurements/Load Flow Bus  LConnTagsString=a|b|c  Phases=ABC  Connectors=on one side  ID=79  Vbase=4160/sqrt(3)  Vref=[1.0 1.0 1.0]  Vangle=[0 -120 120]  VLF=1  VLFb=1  VLFc=1  angleLF=0  angleLFb=0  angleLFc=0
      settings: SourceProductName=Simscape Electrical
  Load Flow Bus128 : powerlib/Measurements/Load Flow Bus  LConnTagsString=a|b|c  Phases=ABC  Connectors=on one side  ID=66  Vbase=4160/sqrt(3)  Vref=[1.0 1.0 1.0]  Vangle=[0 -120 120]  VLF=1  VLFb=1  VLFc=1  angleLF=0  angleLFb=0  angleLFc=0
      settings: SourceProductName=Simscape Electrical
  Load Flow Bus2 : powerlib/Measurements/Load Flow Bus  LConnTagsString=a|b|c  RConnTagsString=a|b|c  Phases=ABC  Connectors=on both sides  ID=36  Vbase=4160/sqrt(3)  Vref=[1.0 1.0]  Vangle=[0 -120]  VLF=1  VLFb=1  VLFc=1  angleLF=0  angleLFb=0  angleLFc=0
      settings: SourceProductName=Simscape Electrical
  Load Flow Bus44 : powerlib/Measurements/Load Flow Bus  LConnTagsString=a|b|c  RConnTagsString=a|b|c  Phases=ABC  Connectors=on both sides  ID=300  Vbase=4160/sqrt(3)  Vref=[1.0 1.0 1.0]  Vangle=[0 -120 120]  VLF=1  VLFb=1  VLFc=1  angleLF=0  angleLFb=0  angleLFc=0
      settings: SourceProductName=Simscape Electrical
  Load Flow Bus45 : powerlib/Measurements/Load Flow Bus  LConnTagsString=a|b|c  Phases=ABC  Connectors=on one side  ID=350  Vbase=4160/sqrt(3)  Vref=[1.0 1.0 1.0]  Vangle=[0 -120 120]  VLF=1  VLFb=1  VLFc=1  angleLF=0  angleLFb=0  angleLFc=0
      settings: SourceProductName=Simscape Electrical
  Load Flow Bus55 : powerlib/Measurements/Load Flow Bus  LConnTagsString=a|b  RConnTagsString=a|b  Phases=AB  Connectors=on both sides  ID=36  Vbase=4160/sqrt(3)  Vref=[1.0 1.0]  Vangle=[0 -120]  VLF=1  VLFb=1  VLFc=1  angleLF=0  angleLFb=0  angleLFc=0
      settings: SourceProductName=Simscape Electrical
  Load Flow Bus68 : powerlib/Measurements/Load Flow Bus  LConnTagsString=a|b|c  Phases=ABC  Connectors=on one side  ID=56  Vbase=4160/sqrt(3)  Vref=[1.0 1.0 1.0]  Vangle=[0 -120 120]  VLF=1  VLFb=1  VLFc=1  angleLF=0  angleLFb=0  angleLFc=0
      settings: SourceProductName=Simscape Electrical
  Load Flow Bus77 : powerlib/Measurements/Load Flow Bus  LConnTagsString=a|b|c  RConnTagsString=a|b|c  Phases=ABC  Connectors=on both sides  ID=95  Vbase=4160/sqrt(3)  Vref=[1.0 1.0 1.0]  Vangle=[0 -120 120]  VLF=1  VLFb=1  VLFc=1  angleLF=0  angleLFb=0  angleLFc=0
      settings: SourceProductName=Simscape Electrical
  Load Flow Bus78 : powerlib/Measurements/Load Flow Bus  LConnTagsString=a|b|c  Phases=ABC  Connectors=on one side  ID=195  Vbase=4160/sqrt(3)  Vref=[1.0 1.0 1.0]  Vangle=[0 -120 120]  VLF=1  VLFb=1  VLFc=1  angleLF=0  angleLFb=0  angleLFc=0
      settings: SourceProductName=Simscape Electrical
  Load Flow Bus84 : powerlib/Measurements/Load Flow Bus  Commented=on  LConnTagsString=a|b|c  Phases=ABC  Connectors=on one side  ID=610  Vbase=480/sqrt(3)  Vref=[1.0 1.0 1.0]  Vangle=[0 -120 120]  VLF=1  VLFb=1  VLFc=1  angleLF=0  angleLFb=0  angleLFc=0
      settings: SourceProductName=Simscape Electrical
  Measurements : Subsystem
  RG1in : powerlib/Measurements/Three-Phase V-I Measurement  VoltageMeasurement=phase-to-ground  SetLabelV=on  LabelV=RG1in  Vpu=off  VpuLL=off  CurrentMeasurement=no  SetLabelI=on  LabelI=I800  Ipu=off  Pbase=100e6  Vbase=24900  OutputType=Complex  PhasorSimulation=on  PSBequivalent=0
      settings: SourceProductName=Simscape Electrical
  RG1out : powerlib/Measurements/Three-Phase V-I Measurement  VoltageMeasurement=phase-to-ground  SetLabelV=on  LabelV=RG1out  Vpu=off  VpuLL=off  CurrentMeasurement=no  SetLabelI=on  LabelI=I800  Ipu=off  Pbase=100e6  Vbase=24900  OutputType=Complex  PhasorSimulation=on  PSBequivalent=0
      settings: SourceProductName=Simscape Electrical
  RG2in : Subsystem
  RG2out : Subsystem
  RG3in : Subsystem
  RG3out : Subsystem
  RG4in : powerlib/Measurements/Three-Phase V-I Measurement  VoltageMeasurement=phase-to-ground  SetLabelV=on  LabelV=RG4in  Vpu=off  VpuLL=off  CurrentMeasurement=no  SetLabelI=on  LabelI=I800  Ipu=off  Pbase=100e6  Vbase=24900  OutputType=Complex  PhasorSimulation=on  PSBequivalent=0
      settings: SourceProductName=Simscape Electrical
  RG4out : powerlib/Measurements/Three-Phase V-I Measurement  VoltageMeasurement=phase-to-ground  SetLabelV=on  LabelV=RG4out  Vpu=off  VpuLL=off  CurrentMeasurement=no  SetLabelI=on  LabelI=I800  Ipu=off  Pbase=100e6  Vbase=24900  OutputType=Complex  PhasorSimulation=on  PSBequivalent=0
      settings: SourceProductName=Simscape Electrical
  Regulator 1 Three Phase Ganged SVR : Subsystem
  Regulator Taps : Subsystem
  Regulator2 : Subsystem
  Regulator3 : Subsystem
  Series RLC Branch1 : powerlib/Elements/Series RLC Branch  LConnTagsString=__new0  RConnTagsString=__new0  BranchType=R  Resistance=.001  Inductance=0  SetiL0=off  InitialCurrent=0  Capacitance=0  Setx0=off  InitialVoltage=0  Measurements=None
      settings: SourceProductName=Simscape Electrical
  Series RLC Branch2 : powerlib/Elements/Series RLC Branch  LConnTagsString=__new0  RConnTagsString=__new0  BranchType=R  Resistance=.001  Inductance=0  SetiL0=off  InitialCurrent=0  Capacitance=0  Setx0=off  InitialVoltage=0  Measurements=None
      settings: SourceProductName=Simscape Electrical
  Series RLC Branch3 : powerlib/Elements/Series RLC Branch  LConnTagsString=__new0  RConnTagsString=__new0  BranchType=R  Resistance=.001  Inductance=0  SetiL0=off  InitialCurrent=0  Capacitance=0  Setx0=off  InitialVoltage=0  Measurements=None
      settings: SourceProductName=Simscape Electrical
  Substation Power : Subsystem
  Three Phase SVR : Subsystem
  Three-Phase Transformer (Two Windings) : powerlib/Elements/Three-Phase Transformer (Two Windings)  Winding1Connection=Delta (D1)  Winding2Connection=Delta (D1)  CoreType=Three single-phase transformers  SetSaturation=off  Hysteresis=off  DataFile='hysteresis'  SetInitialFlux=off  Measurements=None  UNITS=pu  NominalPower=[ 500e3 , 60 ]  Winding1=[4160 0.0127 0.0272]  Winding2=[480 0.0127 0.0272]  Rm=1000  Lm=1000  L0=0.5  Saturation=[ 0,0 ; 0.0024,1.2 ; 1.0,1.52 ]  InitialFluxes=[ 0.8 , -0.8 , 0.7 ]  BreakLoop=on  DiscreteSolver=Trapezoidal iterative  DataType=off  TransfoNumber=1
      settings: SourceProductName=Simscape Electrical
  Three-Phase Breaker1 : powerlib/Elements/Three-Phase Breaker  InitialState=open  SwitchA=off  SwitchB=off  SwitchC=off  SwitchTimes="[1/60  5/60]"  External=off  BreakerResistance=0.01  SnubberResistance=1e6  SnubberCapacitance=inf  Measurements=None
      settings: SourceProductName=Simscape Electrical
  XF1 : powerlib/Measurements/Three-Phase V-I Measurement  VoltageMeasurement=phase-to-ground  SetLabelV=on  LabelV=XF1  Vpu=off  VpuLL=off  CurrentMeasurement=no  SetLabelI=on  LabelI=I65  Ipu=off  Pbase=100e6  Vbase=24900  OutputType=Complex  PhasorSimulation=on  PSBequivalent=0
      settings: SourceProductName=Simscape Electrical
  powergui : powerlib/powergui  Priority=1  SimulationMode=Discrete  SampleTime=Ts  frequency=60  Iterations=50  frequencyindice=0  Pbase=100e6  ErrMax=1e-4  UnitsV=kV  UnitsW=MW  buscounter=0  FunctionMessages=off  echomessages=on  EnableUseOfTLC=off  CurrentSourceSwitches=off  DisableSnubberDevices=off  DisableRonSwitches=off  DisableVfSwitches=off  DisplayEquations=off  AutomaticDiscreteSolvers=off  SolverType=Tustin/Backward Euler (TBE)  Interpol=off  ExternalGateDelay=off  methode=off  Ts=0  x0status=blocks  SPID=off  SwTol=0  HookPort=off  NonlinearTolerance=1e-4  nMaxIteration=100  ContinueOnMaxIteration=off  RestoreLinks=warning  ResistiveCurrentMeasurement=off  Frange=[0:2:500]  Ylog=off  Xlog=on  ShowGrid=off  save=off  variable=ZData  structure=0  ZoomFFT=off  StartTime=0.0  cycles=1  DisplayStyle=1  fundamental=60  FreqAxis=off  MaxFrequency=1000  frequencyindicesteady=1  RmsSteady=1  display=off
      settings: SourceProductName=Simscape Electrical
  tag scope: Reg1=global, Reg2=global, Reg3=global, Reg4=global
  wires:
  Three Phase SVR/1(Tap) -> [Reg4]
  Regulator3/1(Taps) -> [Reg3]
  Regulator2/1(Tap) -> [Reg2]
  Regulator 1 Three Phase Ganged SVR/1(Tap) -> [Reg1]
  connections:
  25-26 7/RConn1 -- 26/LConn1
  25-26 7/LConn2 -- RG3out/RConn2
  25-26 7/LConn1 -- RG3out/RConn1
  26-7 7/RConn2 -- 27/LConn2
  26-7 7/RConn1 -- 27/LConn1
  26-7 7/LConn2 -- 26/RConn2
  26-7 7/LConn1 -- 26/RConn1
  51-151 4/RConn3 -- 151/RConn3
  51-151 4/RConn2 -- 151/RConn2
  51-151 4/RConn1 -- 151/RConn1
  Three Phase SVR/RConn3 -- RG4out/LConn3
  Three Phase SVR/RConn2 -- RG4out/LConn2
  Three Phase SVR/RConn1 -- RG4out/LConn1
  Three Phase SVR/LConn3 -- RG4in/RConn3
  Three Phase SVR/LConn2 -- RG4in/RConn2
  Three Phase SVR/LConn1 -- RG4in/RConn1
  RG3out/LConn2 -- Regulator3/RConn2
  Regulator3/RConn1 -- RG3out/LConn1
  Regulator3/LConn2 -- RG3in/RConn2
  Regulator3/LConn1 -- RG3in/RConn1
  Regulator2/RConn1 -- RG2out/LConn1
  Regulator2/LConn1 -- RG2in/RConn1
  Regulator 1 Three Phase Ganged SVR/RConn3 -- RG1out/LConn3
  Regulator 1 Three Phase Ganged SVR/RConn2 -- RG1out/LConn2
  Regulator 1 Three Phase Ganged SVR/RConn1 -- RG1out/LConn1
  Regulator 1 Three Phase Ganged SVR/LConn3 -- RG1in/RConn3
  Regulator 1 Three Phase Ganged SVR/LConn2 -- RG1in/RConn2
  Regulator 1 Three Phase Ganged SVR/LConn1 -- RG1in/RConn1
  Series RLC Branch2/LConn1 -- 4160 V swing/RConn3
  Series RLC Branch1/LConn1 -- 4160 V swing/RConn2
  Series RLC Branch3/LConn1 -- 4160 V swing/RConn1
  Series RLC Branch2/RConn1 -- 150/LConn3
  Series RLC Branch1/RConn1 -- 150/LConn2
  Series RLC Branch3/RConn1 -- 150/LConn1
  Load Flow Bus2/LConn3 -- 35/RConn3
  Load Flow Bus2/LConn2 -- 35/RConn2
  Load Flow Bus2/LConn1 -- 35/RConn1
  61-610/RConn3 -- XF1/LConn3
  XF1/RConn3 -- Three-Phase Transformer (Two Windings)/LConn3
  RG1out/RConn3 -- 149/LConn3
  RG1out/RConn2 -- 149/LConn2
  RG1out/RConn1 -- 149/LConn1
  RG2out/RConn1 -- 14/LConn1
  160-67 6/RConn3 -- RG4in/LConn3
  160-67 6/RConn2 -- RG4in/LConn2
  160-67 6/RConn1 -- RG4in/LConn1
  RG2in/LConn1 -- 9-14 9/RConn1
  610/RConn3 -- Load Flow Bus84/LConn3
  610/RConn2 -- Load Flow Bus84/LConn2
  610/RConn1 -- Load Flow Bus84/LConn1
  610/LConn3 -- Three-Phase Transformer (Two Windings)/RConn3
  610/LConn2 -- Three-Phase Transformer (Two Windings)/RConn2
  610/LConn1 -- Three-Phase Transformer (Two Windings)/RConn1
  XF1/RConn2 -- Three-Phase Transformer (Two Windings)/LConn2
  XF1/RConn1 -- Three-Phase Transformer (Two Windings)/LConn1
  XF1/LConn2 -- 61-610/RConn2
  XF1/LConn1 -- 61-610/RConn1
  85/RConn1 -- 85 Y PQ/LConn1
  75 Y PQ/LConn1 -- 75/RConn1
  71/RConn1 -- 71 Y PQ/LConn1
  104/LConn1 -- 103-104 11/RConn1
  107/LConn1 -- 106-107 10/RConn1
  114/RConn1 -- 114 Y PQ/LConn1
  111/RConn1 -- 111 Y PQ/LConn1
  87-88 9/RConn1 -- 88/LConn1
  89-90 10/RConn1 -- 90/LConn1
  91-92 11/RConn1 -- 92/LConn1
  96 Y PQ/LConn1 -- 96/RConn1
  17/LConn1 -- 15-17 11/RConn1
  15-16 11/RConn1 -- 16/LConn1
  59 Y PQ/LConn1 -- 59/RConn1
  57-58 10/RConn1 -- 58/LConn1
  36/RConn2 -- Load Flow Bus55/LConn2
  36/LConn2 -- 35-36 8/RConn2
  36/RConn1 -- Load Flow Bus55/LConn1
  37 Y Z/LConn1 -- 37/RConn1
  38-39 10/RConn1 -- 39/LConn1
  41/RConn1 -- 41 Y PQ/LConn1
  43/RConn1 -- 43 Y Z/LConn1
  45-46 9/RConn1 -- 46/LConn1
  32/LConn1 -- 31-32 11/RConn1
  33 Y I/LConn1 -- 33/RConn1
  27/RConn2 -- Load Flow Bus1/RConn2
  27/RConn1 -- Load Flow Bus1/RConn1
  24/LConn1 -- 23-24 11/RConn1
  22/LConn1 -- 21-22 10/RConn1
  20/RConn1 -- 20 Y I/LConn1
  95/RConn3 -- Load Flow Bus77/RConn3
  95/RConn2 -- Load Flow Bus77/RConn2
  95/RConn1 -- Load Flow Bus77/RConn1
  79/RConn3 -- Load Flow Bus117/LConn3
  79/RConn2 -- Load Flow Bus117/LConn2
  79/LConn3 -- 78-79 6/RConn3
  79/LConn2 -- 78-79 6/RConn2
  79/LConn1 -- 78-79 6/RConn1
  151/LConn3 -- 151-1/LConn3
  151/LConn2 -- 151-1/LConn2
  151/LConn1 -- 151-1/LConn1
  300/RConn3 -- Load Flow Bus44/LConn3
  300/RConn2 -- Load Flow Bus44/LConn2
  300/RConn1 -- Load Flow Bus44/LConn1
  450/RConn3 -- Load Flow Bus106/LConn3
  450/RConn2 -- Load Flow Bus106/LConn2
  450/RConn1 -- Load Flow Bus106/LConn1
  450/LConn3 -- 100-450 3/RConn3
  450/LConn2 -- 100-450 3/RConn2
  450/LConn1 -- 100-450 3/RConn1
  56/RConn3 -- Load Flow Bus68/LConn3
  56/RConn1 -- Load Flow Bus68/LConn1
  56/LConn3 -- 55-56 1/RConn3
  56/LConn2 -- 55-56 1/RConn2
  56/LConn1 -- 55-56 1/RConn1
  66/RConn2 -- Load Flow Bus128/LConn2
  66/RConn1 -- Load Flow Bus128/LConn1
  66/LConn3 -- 65-66 12/RConn3
  66/LConn2 -- 65-66 12/RConn2
  66/LConn1 -- 65-66 12/RConn1
  51/RConn3 -- 51-151 4/LConn3
  51/RConn2 -- 51-151 4/LConn2
  51/LConn3 -- 50-51 4/RConn3
  51/LConn2 -- 50-51 4/RConn2
  51/LConn1 -- 50-51 4/RConn1
  48/LConn3 -- 48 Y Z/LConn3
  48 Y Z/LConn2 -- 48/LConn2
  48/LConn1 -- 48 Y Z/LConn1
  12/LConn1 -- 8-12 10/RConn1
  6/RConn1 -- 6 Y Z/LConn1
  4Y PQ/LConn1 -- 4/RConn1
  11/RConn1 -- 11 Y Z/LConn1
  10/LConn1 -- 14-10 9/RConn1
  2/LConn1 -- 1-2 10/RConn1
  RG1in/LConn3 -- 150-1/RConn3
  RG1in/LConn2 -- 150-1/RConn2
  RG1in/LConn1 -- 150-1/RConn1
  1/RConn3 -- 1-7 1/LConn3 -- 1-3 11/LConn1
  1/RConn2 -- 1-7 1/LConn2
  1 Y PQ/LConn1 -- 1-7 1/LConn1 -- 1/RConn1
  Load Flow Bus44/RConn2 -- 300-1/LConn2
  Load Flow Bus44/RConn1 -- 300-1/LConn1
  300-1/RConn3 -- Load Flow Bus45/LConn3
  300-1/RConn2 -- Load Flow Bus45/LConn2
  300-1/RConn1 -- Load Flow Bus45/LConn1
  197/LConn3 -- 97-1/RConn3
  197/LConn2 -- 97-1/RConn2
  197/LConn1 -- 97-1/RConn1
  18-21 2/LConn3 -- 18-135/LConn3 -- 18/RConn3
  18-21 2/LConn2 -- 18-135/LConn2 -- 18/RConn2
  18-21 2/LConn1 -- 18-135/LConn1 -- 18/RConn1 -- 18-19 9/LConn1
  150/RConn3 -- 150-1/LConn3
  150/RConn1 -- 150-1/LConn1
  61/RConn3 -- 61-610/LConn3
  61/RConn2 -- 61-610/LConn2
  61/RConn1 -- 61-610/LConn1
  160-67 6/LConn1 -- 160/RConn1
  160-67 6/LConn2 -- 160/RConn2
  54/LConn1 -- 59-94/LConn1 -- 53-54 1/RConn1 -- 54-57 3/LConn1
  93-95 6/RConn3 -- Three-Phase Breaker1/LConn3 -- 95/LConn3
  93-95 6/RConn2 -- Three-Phase Breaker1/LConn2 -- 95/LConn2 -- 95 Y PQ/LConn1
  93-95 6/RConn1 -- Three-Phase Breaker1/LConn1 -- 95/LConn1
  450-451/LConn3 -- Load Flow Bus106/RConn3
  Load Flow Bus106/RConn2 -- 450-451/LConn2
  Load Flow Bus106/RConn1 -- 450-451/LConn1
  Load Flow Bus44/RConn3 -- 300-1/LConn3
  250/RConn3 -- 250-251/LConn3
  250/RConn2 -- 250-251/LConn2
  250/RConn1 -- 250-251/LConn1
  135/LConn3 -- 18-135/RConn3
  135/LConn2 -- 18-135/RConn2
  135/LConn1 -- 18-135/RConn1
  40/LConn2 -- 35-40 1/RConn2
  40/LConn1 -- 35-40 1/RConn1
  40/LConn3 -- 35-40 1/RConn3
  77/RConn3 -- 77-78 6/LConn3
  77/RConn1 -- 77-78 6/LConn1
  77/RConn2 -- 77-78 6/LConn2
  87/RConn3 -- 87-89 6/LConn3
  87 Y PQ/LConn1 -- 87/RConn2 -- 87-89 6/LConn2
  15/LConn1 -- 34-15 11/RConn1
  64/RConn3 -- 64-65 12/LConn3
  64/RConn2 -- 64-65 12/LConn2
  64/RConn1 -- 64-65 12/LConn1
  110/RConn1 -- 110-112 9/LConn1
  55/LConn3 -- 54-55 1/RConn3
  55/LConn1 -- 54-55 1/RConn1
  55/LConn2 -- 54-55 1/RConn2
  74 Y Z/LConn1 -- 74/LConn1 -- 73-74 11/RConn1
  50/RConn3 -- 50-51 4/LConn3
  50/RConn2 -- 50-51 4/LConn2
  50/RConn1 -- 50-51 4/LConn1
  "30 "/RConn3 -- 30-250 2/LConn3
  "30 "/RConn2 -- 30-250 2/LConn2
  "30 "/RConn1 -- 30-250 2/LConn1
  98/RConn3 -- 98-99 3/LConn3
  98/RConn2 -- 98-99 3/LConn2
  98 Y PQ/LConn1 -- 98/RConn1 -- 98-99 3/LConn1
  57/LConn1 -- 57-60 3/LConn1
  57/LConn3 -- 57-60 3/LConn3
  57/LConn2 -- 57-60 3/LConn2
  7/RConn3 -- 7-8 1/LConn3
  7/RConn2 -- 7-8 1/LConn2
  7/RConn1 -- 7-8 1/LConn1
  93/LConn1 -- 91-93 6/RConn1
  93/LConn3 -- 91-93 6/RConn3
  93/LConn2 -- 91-93 6/RConn2
  81/RConn2 -- 81-82 6/LConn2
  81/RConn1 -- 81-82 6/LConn1
  72/RConn3 -- 72-76 3/LConn3
  72/RConn2 -- 72-76 3/LConn2
  72/RConn1 -- 72-76 3/LConn1
  101/RConn3 -- 101-105 3/LConn3
  101/RConn2 -- 101-105 3/LConn2
  101/RConn1 -- 101-105 3/LConn1
  108/RConn3 -- 108-300 3/LConn3
  108/RConn2 -- 108-300 3/LConn2
  108-109 9/LConn1 -- 108/RConn1 -- 108-300 3/LConn1
  44/RConn3 -- 44-47 1/LConn3
  44/RConn2 -- 44-47 1/LConn2
  25/RConn3 -- 25-28 2/LConn3
  25/RConn2 -- 25-28 2/LConn2
  25/RConn1 -- 25-28 2/LConn1
  160-67 6/LConn3 -- 160/RConn3
  13-152/RConn3 -- 152/LConn3
  13-152/RConn2 -- 152/LConn2
  13-152/RConn1 -- 152/LConn1
  65 D Z/LConn1 -- 64-65 12/RConn1 -- 65/LConn1
  65 D Z/LConn3 -- 64-65 12/RConn3 -- 65/LConn3
  55 Y Z/LConn1 -- 55/RConn1 -- 55-56 1/LConn1
  55/RConn2 -- 55-56 1/LConn2
  55/RConn3 -- 55-56 1/LConn3
  51 Y PQ/LConn1 -- 51-151 4/LConn1 -- 51/RConn1
  21/RConn1 -- 21-23 2/LConn1
  33/LConn1 -- 27-33 9/RConn1
  72/LConn3 -- 67-72 3/RConn3
  56 Y PQ/LConn1 -- Load Flow Bus68/LConn2 -- 56/RConn2
  25/LConn3 -- RG3in/LConn2 -- 23-25 2/RConn3
  74-75 11/RConn1 -- 75/LConn1
  47 Y I/LConn2 -- 47/LConn2 -- 47-48 4/RConn2
  72-73 11/RConn1 -- 73/LConn1 -- 73 Y PQ/LConn1
  70-71 1/RConn1 -- 71/LConn1
  29/LConn3 -- 28-29 2/RConn3
  70 Y PQ/LConn1 -- 70/RConn1 -- 70-71 1/LConn1
  17 Y PQ/LConn1 -- 17/RConn1
  21-22 10/LConn1 -- 21/RConn2 -- 21-23 2/LConn2
  70/LConn1 -- 69-70 9/RConn1
  54/RConn3 -- 54-55 1/LConn3
  135-35 4/RConn1 -- 35/LConn1 -- 35-40 1/LConn1
  60-61 5/LConn2 -- 60/LConn2 -- 60-1/LConn2 -- 60-62 12/LConn2
  12 Y PQ/LConn1 -- 12/RConn1
  7/LConn2 -- 1-7 1/RConn2
  67/LConn2 -- 67-72 3/LConn2
  89/LConn2 -- 87-89 6/RConn2
  87/LConn2 -- 86-87 6/RConn2
  8/RConn3 -- 8-13 1/LConn3
  13/LConn1 -- 8-13 1/RConn1
  8/RConn2 -- 8-13 1/LConn2
  8-9 9/LConn1 -- 8/LConn1 -- 7-8 1/RConn1
  93/RConn2 -- 93-95 6/LConn2
  89-90 10/LConn1 -- 89/RConn2 -- 89-91 6/LConn2
  16/RConn1 -- 16 Y PQ/LConn1
  5/LConn1 -- 3-5 11/RConn1
  3-4 11/RConn1 -- 4/LConn1
  13-34 11/LConn1 -- 13/LConn3 -- 8-13 1/RConn3
  9-14 9/LConn1 -- 9/RConn1 -- 9 Y PQ/LConn1
  13-18 2/LConn1 -- 13/RConn1 -- 13-152/LConn1
  13-18 2/LConn3 -- 13/RConn3 -- 13-152/LConn3
  18/LConn2 -- 13-18 2/RConn2
  18/LConn1 -- 13-18 2/RConn1
  18/LConn3 -- 13-18 2/RConn3
  10 Y I/LConn1 -- 10/RConn1
  14-11 9/LConn1 -- 14-10 9/LConn1 -- 14/RConn1
  8/RConn1 -- 8-13 1/LConn1
  1-7 1/RConn1 -- 7/LConn1 -- 7 Y PQ/LConn1
  7/LConn3 -- 1-7 1/RConn3
  47/RConn1 -- 47-49 4/LConn1
  15-17 11/LConn1 -- 15/RConn1 -- 15-16 11/LConn1
  42/RConn1 -- 42-44 1/LConn1
  14-11 9/RConn1 -- 11/LConn1
  34/LConn1 -- 13-34 11/RConn1
  53/LConn3 -- 52-53 1/RConn3
  3/LConn1 -- 1-3 11/RConn1
  57-58 10/LConn1 -- 57/RConn2 -- 54-57 3/RConn2
  21/LConn3 -- 18-21 2/RConn3
  73/RConn1 -- 73-74 11/LConn1
  74/RConn1 -- 74-75 11/LConn1
  53/RConn1 -- 53-54 1/LConn1
  52/RConn2 -- 52-53 1/LConn2
  53/RConn3 -- 53-54 1/LConn3
  53/LConn2 -- 52-53 1/RConn2
  21/LConn2 -- 18-21 2/RConn2
  35 D PQ/LConn1 -- Load Flow Bus2/RConn1 -- 35-36 8/LConn1
  53 Y PQ/LConn1 -- 52-53 1/RConn1 -- 53/LConn1
  52/RConn3 -- 52-53 1/LConn3
  53/RConn2 -- 53-54 1/LConn2
  135-35 4/RConn2 -- 35/LConn2 -- 35-40 1/LConn2
  65/RConn2 -- 65-66 12/LConn2
  63/LConn3 -- 62-63 12/RConn3
  58 Y I/LConn1 -- 58-59 10/LConn1 -- 58/RConn1
  5-6 11/RConn1 -- 6/LConn1
  19/RConn1 -- 19-20 9/LConn1
  60/RConn1 -- 57-60 3/RConn1
  5-6 11/LConn1 -- 5/RConn1 -- 5 Y I/LConn1
  63/RConn1 -- 63-64 12/LConn1
  63/RConn2 -- 63-64 12/LConn2
  69 Y PQ/LConn1 -- 69-70 9/LConn1 -- 69/RConn1
  62/LConn1 -- 60-62 12/RConn1
  24 Y PQ/LConn1 -- 24/RConn1
  29/LConn2 -- 28-29 2/RConn2
  57/RConn1 -- 54-57 3/RConn1
  29/RConn1 -- 29-30 2/LConn1
  60-61 5/LConn3 -- 60/LConn3 -- 60-1/LConn3 -- 60-62 12/LConn3
  2 Y PQ/LConn1 -- 2/RConn1
  98/LConn2 -- 97-98 3/RConn2
  63/RConn3 -- 63-64 12/LConn3
  13/LConn2 -- 8-13 1/RConn2
  8-12 10/LConn1 -- 8/LConn2 -- 7-8 1/RConn2
  42-43 10/LConn1 -- 42/RConn2 -- 42-44 1/LConn2
  3-4 11/LConn1 -- 3/RConn1 -- 3-5 11/LConn1
  1-2 10/LConn1 -- 149-1 1/RConn2 -- 1/LConn2
  13-18 2/LConn2 -- 13/RConn2 -- 13-152/LConn2
  9/LConn1 -- 8-9 9/RConn1
  8/LConn3 -- 7-8 1/RConn3
  72-76 3/RConn1 -- 76/LConn1 -- 76-77 6/LConn1
  52/RConn1 -- 52-53 1/LConn1
  40-41 11/LConn1 -- 40/RConn3 -- 40-42 1/LConn3
  28/RConn3 -- 28-29 2/LConn3
  38 Y I/LConn1 -- 38/RConn1 -- 38-39 10/LConn1
  57/RConn3 -- 54-57 3/RConn3
  40-41 11/RConn1 -- 41/LConn1
  60/RConn2 -- 57-60 3/RConn2
  60 Y PQ/LConn1 -- 60/LConn1 -- 60-1/LConn1 -- 60-61 5/LConn1 -- 60-62 12/LConn1
  21/LConn1 -- 18-21 2/RConn1
  23-24 11/LConn1 -- 23/RConn3 -- 23-25 2/LConn3
  29/RConn2 -- 29-30 2/LConn2
  "30 "/LConn1 -- 29-30 2/RConn1
  44-45 9/LConn1 -- 44/RConn1 -- 44-47 1/LConn1
  62/LConn2 -- 60-62 12/RConn2
  64/LConn1 -- 63-64 12/RConn1
  67-97 3/RConn2 -- 97/LConn2
  29/RConn3 -- 29-30 2/LConn3
  67/RConn2 -- 67-97 3/LConn2 -- RG4out/RConn2
  28-29 2/RConn1 -- 29/LConn1 -- 29 Y Z/LConn1
  47 Y I/LConn3 -- 47/LConn3 -- 47-48 4/RConn3
  72-76 3/RConn2 -- 76/LConn2 -- 76-77 6/LConn2
  72-76 3/RConn3 -- 76/LConn3 -- 76-77 6/LConn3
  60/RConn3 -- 57-60 3/RConn3
  28/RConn1 -- 28-29 2/LConn1
  28/RConn2 -- 28-29 2/LConn2
  63/LConn2 -- 62-63 12/RConn2
  53-54 1/RConn3 -- 54/LConn3 -- 54-57 3/LConn3
  22 Y Z/LConn1 -- 22/RConn1
  49/RConn3 -- 49-50 4/LConn3
  23/LConn2 -- 21-23 2/RConn2
  67-68 9/LConn1 -- 67-97 3/LConn1 -- RG4out/RConn1 -- 67/RConn1
  62/RConn3 -- 62-63 12/LConn3
  45/RConn1 -- 45-46 9/LConn1
  49 Y PQ/LConn1 -- 49/LConn1 -- 47-49 4/RConn1
  30 Y PQ/LConn1 -- "30 "/LConn3 -- 29-30 2/RConn3
  54/RConn1 -- 54-55 1/LConn1
  23/LConn3 -- 21-23 2/RConn3
  250/LConn1 -- 30-250 2/RConn1
  27-33 9/LConn1 -- Load Flow Bus1/LConn1
  31/LConn1 -- 26-31 11/RConn1
  40/RConn1 -- 40-42 1/LConn1
  23/RConn2 -- 23-25 2/LConn2
  65/RConn3 -- 65-66 12/LConn3
  66 Y PQ/LConn1 -- Load Flow Bus128/LConn3 -- 66/RConn3
  67-72 3/LConn1 -- 67/LConn1
  69/LConn1 -- 68-69 9/RConn1
  "30 "/LConn2 -- 29-30 2/RConn2
  62 Y Z/LConn1 -- 62/LConn3 -- 60-62 12/RConn3
  23/LConn1 -- 21-23 2/RConn1
  19 Y PQ/LConn1 -- 19/LConn1 -- 18-19 9/RConn1
  59/LConn1 -- 58-59 10/RConn1
  72/LConn1 -- 67-72 3/RConn1
  25/LConn2 -- 23-25 2/RConn2
  47-48 4/LConn2 -- 48/RConn2 -- 44-47 1/RConn2
  68/LConn1 -- 67-68 9/RConn1
  49/RConn1 -- 49-50 4/LConn1
  65/RConn1 -- 65-66 12/LConn1
  47-48 4/LConn1 -- 48/RConn1 -- 44-47 1/RConn1
  63 Y PQ/LConn1 -- 63/LConn1 -- 62-63 12/RConn1
  28/LConn3 -- 25-28 2/RConn3
  21/RConn3 -- 21-23 2/LConn3
  62/RConn2 -- 62-63 12/LConn2
  46/RConn1 -- 46 Y PQ/LConn1
  47 Y I/LConn1 -- 47/LConn1 -- 47-48 4/RConn1
  67/LConn3 -- 72-73 11/LConn1 -- 67-72 3/LConn3
  62/RConn1 -- 62-63 12/LConn1
  64 Y I/LConn1 -- 64/LConn2 -- 63-64 12/RConn2
  47-48 4/LConn3 -- 48/RConn3 -- 44-47 1/RConn3
  28/LConn2 -- 25-28 2/RConn2
  26-31 11/LConn1 -- 25-26 7/RConn2 -- 26/LConn2
  28 Y I/LConn1 -- 28/LConn1 -- 25-28 2/RConn1
  31 Y PQ/LConn1 -- 31/RConn1 -- 31-32 11/LConn1
  250/LConn2 -- 30-250 2/RConn2
  34-15 11/LConn1 -- 34/RConn1 -- 34 Y Z/LConn1
  35-40 1/LConn3 -- 35/LConn3 -- 135-35 4/RConn3
  37/LConn1 -- 36-37 9/RConn1
  36-38 10/LConn1 -- Load Flow Bus55/RConn2
  38/LConn1 -- 36-38 10/RConn1
  67-97 3/RConn1 -- 97/LConn1
  250/LConn3 -- 30-250 2/RConn3
  32 Y PQ/LConn1 -- 32/RConn1
  50/LConn1 -- 49-50 4/RConn1
  42/LConn3 -- 40-42 1/RConn3
  42/LConn2 -- 40-42 1/RConn2
  44/LConn3 -- 42-44 1/RConn3
  44/LConn2 -- 42-44 1/RConn2
  68 Y PQ/LConn1 -- 68/RConn1 -- 68-69 9/LConn1
  44/LConn1 -- 42-44 1/RConn1
  42-43 10/RConn1 -- 43/LConn1
  42 Y PQ/LConn1 -- 42/LConn1 -- 40-42 1/RConn1
  47/RConn3 -- 47-49 4/LConn3
  42/RConn3 -- 42-44 1/LConn3
  39/RConn1 -- 39 Y PQ/LConn1
  65 D Z/LConn2 -- 64-65 12/RConn2 -- 65/LConn2
  40/RConn2 -- 40-42 1/LConn2
  50/LConn2 -- 49-50 4/RConn2
  50 Y PQ/LConn1 -- 50/LConn3 -- 49-50 4/RConn3
  67-97 3/RConn3 -- 97/LConn3
  45 Y I/LConn1 -- 45/LConn1 -- 44-45 9/RConn1
  23/RConn1 -- 23-25 2/LConn1
  67/RConn3 -- 67-97 3/LConn3 -- RG4out/RConn3
  19-20 9/RConn1 -- 20/LConn1
  35 D PQ/RConn1 -- Load Flow Bus2/RConn2 -- 35-36 8/LConn2
  72/LConn2 -- 67-72 3/RConn2
  54/RConn2 -- 54-55 1/LConn2
  25/LConn1 -- RG3in/LConn1 -- 23-25 2/RConn1
  49 Y PQ/LConn3 -- 49/LConn3 -- 47-49 4/RConn3
  49 Y PQ/LConn2 -- 49/LConn2 -- 47-49 4/RConn2
  49/RConn2 -- 49-50 4/LConn2
  47/RConn2 -- 47-49 4/LConn2
  64/LConn3 -- 63-64 12/RConn3
  36/LConn1 -- 35-36 8/RConn1 -- 36-37 9/LConn1
  53-54 1/RConn2 -- 54/LConn2 -- 54-57 3/LConn2
  Ground7/LConn1 -- 10 Y I/RConn1
  250-251/RConn2 -- Load Flow Bus10/LConn2
  Ground5/LConn1 -- 7 Y PQ/RConn1
  Ground4/LConn1 -- 5 Y I/RConn1
  Ground1/LConn1 -- 2 Y PQ/RConn1
  86/LConn1 -- 76-86 3/RConn1
  61/LConn3 -- 60-61 5/RConn3
  Ground6/LConn1 -- 9 Y PQ/RConn1
  94/LConn1 -- 59-94/RConn1
  450-451/RConn2 -- Load Flow Bus107/LConn2
  Ground8/LConn1 -- 11 Y Z/RConn1
  Ground3/LConn1 -- 6 Y Z/RConn1
  78/LConn2 -- 77-78 6/RConn2
  78/LConn1 -- 77-78 6/RConn1
  Load Flow Bus78/LConn1 -- Three-Phase Breaker1/RConn1
  76 DI/LConn3 -- 76/RConn3 -- 76-86 3/LConn3
  86/LConn2 -- 76-86 3/RConn2
  61/LConn2 -- 60-61 5/RConn2
  Load Flow Bus78/LConn3 -- Three-Phase Breaker1/RConn3
  Ground/LConn1 -- 1 Y PQ/RConn1
  Load Flow Bus78/LConn2 -- Three-Phase Breaker1/RConn2
  Ground9/LConn1 -- 12 Y PQ/RConn1
  Ground10/LConn1 -- 16 Y PQ/RConn1
  Ground11/LConn1 -- 17 Y PQ/RConn1
  Ground12/LConn1 -- 19 Y PQ/RConn1
  Ground13/LConn1 -- 20 Y I/RConn1
  Ground14/LConn1 -- 22 Y Z/RConn1
  Ground15/LConn1 -- 24 Y PQ/RConn1
  Ground16/LConn1 -- 28 Y I/RConn1
  Ground17/LConn1 -- 29 Y Z/RConn1
  Ground18/LConn1 -- 30 Y PQ/RConn1
  Ground19/LConn1 -- 31 Y PQ/RConn1
  Ground20/LConn1 -- 32 Y PQ/RConn1
  Ground21/LConn1 -- 33 Y I/RConn1
  Ground22/LConn1 -- 34 Y Z/RConn1
  Ground23/LConn1 -- 37 Y Z/RConn1
  Ground24/LConn1 -- 38 Y I/RConn1
  Ground25/LConn1 -- 39 Y PQ/RConn1
  Ground26/LConn1 -- 41 Y PQ/RConn1
  Ground27/LConn1 -- 42 Y PQ/RConn1
  Ground28/LConn1 -- 43 Y Z/RConn1
  Ground29/LConn1 -- 45 Y I/RConn1
  Ground30/LConn1 -- 46 Y PQ/RConn1
  Ground31/LConn1 -- 50 Y PQ/RConn1
  Ground32/LConn1 -- 51 Y PQ/RConn1
  Ground33/LConn1 -- 52 Y PQ/RConn1
  Ground34/LConn1 -- 53 Y PQ/RConn1
  Ground35/LConn1 -- 55 Y Z/RConn1
  Ground36/LConn1 -- 56 Y PQ/RConn1
  Ground37/LConn1 -- 58 Y I/RConn1
  Ground38/LConn1 -- 59 Y PQ/RConn1
  Ground39/LConn1 -- 60 Y PQ/RConn1
  Ground40/LConn1 -- 62 Y Z/RConn1
  Ground41/LConn1 -- 63 Y PQ/RConn1
  Ground42/LConn1 -- 64 Y I/RConn1
  Ground43/LConn1 -- 66 Y PQ/RConn1
  Ground44/LConn1 -- 68 Y PQ/RConn1
  Ground45/LConn1 -- 69 Y PQ/RConn1
  Ground46/LConn1 -- 70 Y PQ/RConn1
  Ground47/LConn1 -- 71 Y PQ/RConn1
  Ground48/LConn1 -- 73 Y PQ/RConn1
  Ground49/LConn1 -- 74 Y Z/RConn1
  Ground50/LConn1 -- 75 Y PQ/RConn1
  Ground51/LConn1 -- 77 Y PQ/RConn1
  Ground52/LConn1 -- 79 Y Z/RConn1
  Ground53/LConn1 -- 80 Y PQ/RConn1
  Ground54/LConn1 -- 82 Y PQ/RConn1
  Ground55/LConn1 -- 83 Y PQ/RConn1
  Ground56/LConn1 -- 84 Y PQ/RConn1
  Ground57/LConn1 -- 85 Y PQ/RConn1
  Ground58/LConn1 -- 86 Y PQ/RConn1
  Ground59/LConn1 -- 87 Y PQ/RConn1
  Ground60/LConn1 -- 88 Y PQ/RConn1
  Ground61/LConn1 -- 90 Y I/RConn1
  Ground62/LConn1 -- 92 Y PQ/RConn1
  Ground63/LConn1 -- 94 Y PQ/RConn1
  Ground64/LConn1 -- 95 Y PQ/RConn1
  Ground65/LConn1 -- 96 Y PQ/RConn1
  Ground66/LConn1 -- 98 Y PQ/RConn1
  Ground67/LConn1 -- 99 Y PQ/RConn1
  Ground68/LConn1 -- 100 Y Z/RConn1
  Ground69/LConn1 -- 102 Y Z/RConn1
  Ground70/LConn1 -- 103 Y PQ/RConn1
  Ground71/LConn1 -- 104 Y PQ/RConn1
  Ground72/LConn1 -- 106 Y PQ/RConn1
  Ground73/LConn1 -- 107 Y PQ/RConn1
  Ground74/LConn1 -- 109 Y PQ/RConn1
  Ground75/LConn1 -- 111 Y PQ/RConn1
  Ground76/LConn1 -- 112 Y I/RConn1
  Ground77/LConn1 -- 113 Y Z/RConn1
  Ground78/LConn1 -- 114 Y PQ/RConn1
  83/RConn1 -- 83 Y CAP/LConn1
  83/RConn2 -- 83 Y CAP/LConn2
  83/RConn3 -- 83 Y CAP/LConn3
  Ground79/LConn1 -- 88 Y CAP/RConn1
  Ground80/LConn1 -- 90 Y CAP/RConn1
  Ground81/LConn1 -- 92 Y CAP/RConn1
  149-1 1/RConn3 -- 1/LConn3
  149-1 1/LConn3 -- 149/RConn3
  101/LConn2 -- 197-101 3/RConn2
  76 DI/LConn2 -- 76/RConn2 -- 76-86 3/LConn2
  78/LConn3 -- 77-78 6/RConn3
  100/RConn1 -- 100-450 3/LConn1
  78-80 6/LConn1 -- 78/RConn1 -- 78-79 6/LConn1
  100/LConn1 -- 99-100 3/RConn1
  78-80 6/LConn3 -- 78/RConn3 -- 78-79 6/LConn3
  100/LConn2 -- 99-100 3/RConn2
  100/LConn3 -- 99-100 3/RConn3
  99 Y PQ/LConn1 -- 99/RConn2 -- 99-100 3/LConn2
  77/LConn3 -- 76-77 6/RConn3
  76-77 6/RConn2 -- 77/LConn2 -- 77 Y PQ/LConn1
  77/LConn1 -- 76-77 6/RConn1
  149-1 1/LConn2 -- 149/RConn2
  149-1 1/RConn1 -- 1/LConn1
  101/LConn3 -- 197-101 3/RConn3
  149-1 1/LConn1 -- 149/RConn1
  135/RConn3 -- 135-35 4/LConn3
  52 Y PQ/LConn1 -- 152-52 1/RConn1 -- 52/LConn1
  135/RConn2 -- 135-35 4/LConn2
  135/RConn1 -- 135-35 4/LConn1
  52/LConn2 -- 152-52 1/RConn2
  113-114 9/RConn1 -- 114/LConn1
  113 Y Z/LConn1 -- 113/RConn1 -- 113-114 9/LConn1
  52/LConn3 -- 152-52 1/RConn3
  113/LConn1 -- 112-113 9/RConn1
  152/RConn1 -- 152-52 1/LConn1
  112 Y I/LConn1 -- 112/RConn1 -- 112-113 9/LConn1
  112/LConn1 -- 110-112 9/RConn1
  152/RConn2 -- 152-52 1/LConn2
  110-111 9/LConn1 -- 111/LConn1
  152/RConn3 -- 152-52 1/LConn3
  109-110 9/RConn1 -- 110/LConn1 -- 110-111 9/RConn1
  109-110 9/LConn1 -- 109/RConn1 -- 109 Y PQ/LConn1
  450-451/RConn3 -- Load Flow Bus107/LConn3
  250-251/RConn3 -- Load Flow Bus10/LConn3
  300/LConn3 -- 151-1/RConn3 -- 108-300 3/RConn3
  300/LConn2 -- 151-1/RConn2 -- 108-300 3/RConn2
  300/LConn1 -- 151-1/RConn1 -- 108-300 3/RConn1
  109/LConn1 -- 108-109 9/RConn1
  107 Y PQ/LConn1 -- 107/RConn1
  106 Y PQ/LConn1 -- 106/RConn1 -- 106-107 10/LConn1
  61/LConn1 -- 60-61 5/RConn1
  105-108 3/LConn2 -- 105/RConn2 -- 105-106 10/LConn1
  105/RConn3 -- 105-108 3/LConn3
  105/RConn1 -- 105-108 3/LConn1
  108/LConn3 -- 105-108 3/RConn3
  108/LConn2 -- 105-108 3/RConn2
  108/LConn1 -- 105-108 3/RConn1
  106/LConn1 -- 105-106 10/RConn1
  60-1/RConn1 -- 160/LConn1
  105/LConn2 -- 101-105 3/RConn2
  60-1/RConn2 -- 160/LConn2
  101-102 11/LConn1 -- 105/LConn3 -- 101-105 3/RConn3
  60-1/RConn3 -- 160/LConn3
  105/LConn1 -- 101-105 3/RConn1
  103 Y PQ/LConn1 -- 103/RConn1 -- 103-104 11/LConn1
  104 Y PQ/LConn1 -- 104/RConn1
  197/RConn2 -- 197-101 3/LConn2
  103/LConn1 -- 102-103 11/RConn1
  102-103 11/LConn1 -- 102/RConn1 -- 102 Y Z/LConn1
  197/RConn3 -- 197-101 3/LConn3
  102/LConn1 -- 101-102 11/RConn1
  101/LConn1 -- 197-101 3/RConn1
  100 Y Z/LConn1 -- 100/RConn3 -- 100-450 3/LConn3
  100/RConn2 -- 100-450 3/LConn2
  92 Y PQ/LConn1 -- 92/RConn1 -- 92 Y CAP/LConn1
  91-92 11/LConn1 -- 91/RConn3 -- 91-93 6/LConn3
  Ground2/LConn1 -- 4Y PQ/RConn1
  91/LConn3 -- 89-91 6/RConn3
  91/LConn2 -- 89-91 6/RConn2
  91/LConn1 -- 89-91 6/RConn1
  93-94 9/LConn1 -- 93/RConn1 -- 93-95 6/LConn1
  89/RConn3 -- 89-91 6/LConn3
  89/RConn1 -- 89-91 6/LConn1
  90 Y CAP/LConn1 -- 90/RConn1 -- 90 Y I/LConn1
  89/LConn3 -- 87-89 6/RConn3
  89/LConn1 -- 87-89 6/RConn1
  87-88 9/LConn1 -- 87/RConn1 -- 87-89 6/LConn1
  450-451/RConn1 -- Load Flow Bus107/LConn1
  88 Y CAP/LConn1 -- 88/RConn1 -- 88 Y PQ/LConn1
  95-96 10/LConn1 -- Load Flow Bus77/LConn2
  87/LConn3 -- 86-87 6/RConn3
  87/LConn1 -- 86-87 6/RConn1
  93/RConn3 -- 93-95 6/LConn3
  86/RConn3 -- 86-87 6/LConn3
  86 Y PQ/LConn1 -- 86/RConn2 -- 86-87 6/LConn2
  98/LConn1 -- 97-98 3/RConn1
  150/RConn2 -- 150-1/LConn2
  86/RConn1 -- 86-87 6/LConn1
  96/LConn1 -- 95-96 10/RConn1
  83 Y PQ/LConn1 -- 83/LConn3 -- 82-83 6/RConn3
  98/LConn3 -- 97-98 3/RConn3
  83/LConn2 -- 82-83 6/RConn2
  83/LConn1 -- 82-83 6/RConn1
  82/RConn3 -- 82-83 6/LConn3
  82/RConn2 -- 82-83 6/LConn2
  82 Y PQ/LConn1 -- 82/RConn1 -- 82-83 6/LConn1
  84-85 11/RConn1 -- 85/LConn1
  84/RConn1 -- 84-85 11/LConn1
  99/LConn1 -- 98-99 3/RConn1
  84 Y PQ/LConn1 -- 84/LConn1 -- 81-84 11/RConn1
  250-251/RConn1 -- Load Flow Bus10/LConn1
  99/LConn2 -- 98-99 3/RConn2
  82/LConn3 -- 81-82 6/RConn3
  82/LConn2 -- 81-82 6/RConn2
  99/LConn3 -- 98-99 3/RConn3
  82/LConn1 -- 81-82 6/RConn1
  81-82 6/LConn3 -- 81/RConn3 -- 81-84 11/LConn1
  99/RConn1 -- 99-100 3/LConn1
  76 DI/LConn1 -- 76/RConn1 -- 76-86 3/LConn1
  91/RConn1 -- 91-93 6/LConn1
  81/LConn3 -- 80-81 6/RConn3
  91/RConn2 -- 91-93 6/LConn2
  81/LConn2 -- 80-81 6/RConn2
  81/LConn1 -- 80-81 6/RConn1
  80/RConn3 -- 80-81 6/LConn3
  94 Y PQ/LConn1 -- 94/RConn1 -- 93-94 9/RConn1
  80 Y PQ/LConn1 -- 80/RConn2 -- 80-81 6/LConn2
  80/RConn1 -- 80-81 6/LConn1
  80/LConn3 -- 78-80 6/RConn3
  80/LConn2 -- 78-80 6/RConn2
  97-98 3/LConn1 -- 97-1/LConn1 -- 97/RConn1
  97/RConn3 -- 97-1/LConn3 -- 97-98 3/LConn3
  97-98 3/LConn2 -- 97-1/LConn2 -- 97/RConn2
  197/RConn1 -- 197-101 3/LConn1
  99/RConn3 -- 99-100 3/LConn3
  86/LConn3 -- 76-86 3/RConn3
  79 Y Z/LConn1 -- Load Flow Bus117/LConn1 -- 79/RConn1
  78-80 6/LConn2 -- 78/RConn2 -- 78-79 6/LConn2
  80/LConn1 -- 78-80 6/RConn1
